simulink model "three_b_attitude_control_rotationMatrix"  (R2021a)
settings: Solver=ode23t  StartTime=0.0  StopTime=100  RelTol=1e-5
undefined symbols (not defined in the file): eul_init, g, I, km, kt, L, m, pm_0, sigbuilder_block, thrust_max, TQ_max_per_motor, Vb_init, Vm_0, wb_init, Xe_init, xme_0
libraries: simulink_extras x18, sharedtransform x3, simulink x1
(part 1 of 2)
settings Model: Creator=Petronas-Tareq  LastModifiedBy=Petronas-Tareq

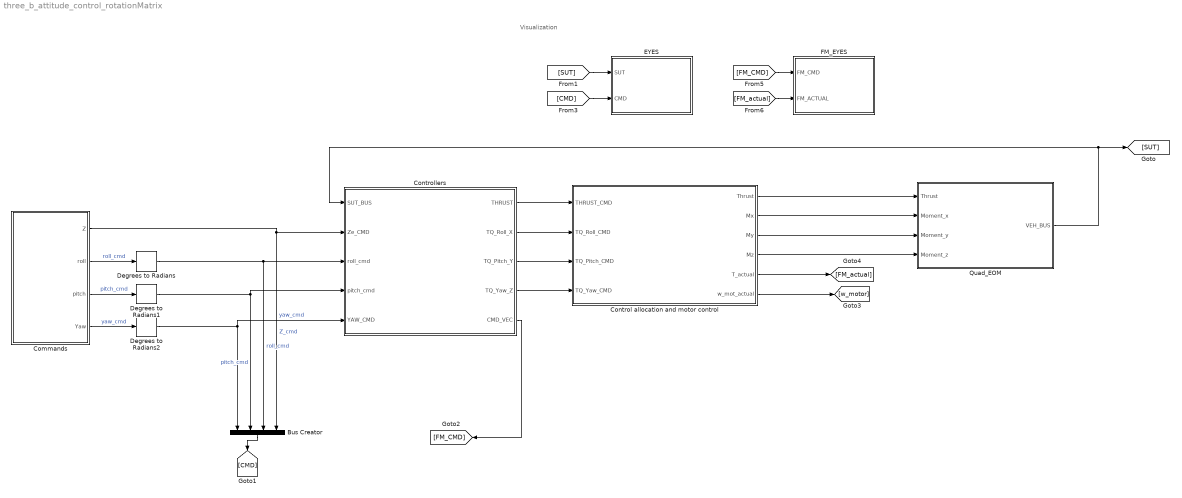
== system three_b_attitude_control_rotationMatrix ==
  note: Visualization
  Bus Creator : BusCreator  Inputs=4
  Commands : Subsystem  Variant=on  VariantControlMode=label  LabelModeActiveChoice=Choice_5
  Control allocation and motor control : Subsystem  Variant=on  VariantControlMode=label  LabelModeActiveChoice=Choice2
      mask Display: image('$imagefile'); % Use "Edit Image" on toolstrip to change.
  Controllers : Subsystem
      mask Display: image('$imagefile'); % Use "Edit Image" on toolstrip to change.
  Degrees to Radians : simulink_extras/Transformations/Degrees to Radians
  Degrees to Radians1 : simulink_extras/Transformations/Degrees to Radians
  Degrees to Radians2 : simulink_extras/Transformations/Degrees to Radians
  EYES : Subsystem
  FM_EYES : Subsystem
  Quad_EOM : Subsystem
      mask Display: image('$imagefile'); % Use "Edit Image" on toolstrip to change.
  wires:
  [FM_CMD] -> FM_EYES/1(FM_CMD)
  Controllers/5(CMD_VEC) -> [FM_CMD]
  [FM_actual] -> FM_EYES/2(FM_ACTUAL)
  Commands/1(Z) -> Bus Creator/4, Controllers/2(Ze_CMD)  "Z_cmd"
  Degrees to Radians/1 -> Bus Creator/3, Controllers/3(roll_cmd)  "roll_cmd"
  Degrees to Radians2/1 -> Bus Creator/1, Controllers/5(YAW_CMD)  "yaw_cmd"
  [SUT] -> EYES/1(SUT)
  [CMD] -> EYES/2(CMD)
  Bus Creator/1 -> [CMD]
  Degrees to Radians1/1 -> Bus Creator/2, Controllers/4(pitch_cmd)  "pitch_cmd"
  Commands/2(roll) -> Degrees to Radians/1  "roll_cmd"
  Commands/3(pitch) -> Degrees to Radians1/1  "pitch_cmd"
  Commands/4(Yaw) -> Degrees to Radians2/1  "yaw_cmd"
  Controllers/1(THRUST) -> Control allocation and motor control/1(THRUST_CMD)
  Controllers/2(TQ_Roll_X) -> Control allocation and motor control/2(TQ_Roll_CMD)
  Controllers/3(TQ_Pitch_Y) -> Control allocation and motor control/3(TQ_Pitch_CMD)
  Controllers/4(TQ_Yaw_Z) -> Control allocation and motor control/4(TQ_Yaw_CMD)
  Control allocation and motor control/1(Thrust) -> Quad_EOM/1(Thrust)
  Control allocation and motor control/2(Mx) -> Quad_EOM/2(Moment_x)
  Control allocation and motor control/3(My) -> Quad_EOM/3(Moment_y)
  Control allocation and motor control/4(Mz) -> Quad_EOM/4(Moment_z)
  Control allocation and motor control/5(T_actual) -> [FM_actual]
  Control allocation and motor control/6(w_mot_actual) -> [w_motor]
  Quad_EOM/1(VEH_BUS) -> [SUT], Controllers/1(SUT_BUS)

== system three_b_attitude_control_rotationMatrix/Commands ==
  note: 1) Add Subsystem or Model blocks as valid variant choices.
      | 2) You cannot connect blocks at this level. At simulation, connectivity is automatically
      | determined, based on the active variant and port name matching.
  "Altitude " : Subsystem  Tag=STV Subsys  LoadFcn=sigbuilder_block('load');  StartFcn=sigbuilder_block('start');  StopFcn=sigbuilder_block('stop');  ClipboardFcn=sigbuilder_block('clipboard');  VariantControl=Choice_1  mask(Sigbuilder block){tuvar=[0:10]}
      mask help: Simulink:masks:SigbuilderBlock_MD
      mask init:
      | if ~strcmp(get_param(bdroot(gcbh),'SimulationStatus'),'stopped') tuvar = sigbuilder_block('maskInit'); end
      settings: CopyFcn=sigbuilder_block('copy');  DeleteFcn=sigbuilder_block('delete');  ModelCloseFcn=sigbuilder_block('modelClose');  PreSaveFcn=sigbuilder_block('preSave');  PauseFcn=sigbuilder_block('pause');  ContinueFcn=sigbuilder_block('continue');  NameChangeFcn=sigbuilder_block('namechange');  OpenFcn=sigbuilder_block('open',[200.1 155.1 551.4 400.5 ]);  CloseFcn=sigbuilder_block('close');
      mask Display: plot(0, 0, 100, 100,[2, 2, 32, 32, 2], [68, 8, 8, 68, 68],[32, 2], [38, 38], [32, 19, 2],[53, 60, 44], [32, 17, 17, 2],[16, 16, 31, 31]);txt = getActiveGroup(gcbh);text(2, 100, txt,'verticalAlignment', 'top');
  Ground : Subsystem  Tag=STV Subsys  LoadFcn=sigbuilder_block('load');  StartFcn=sigbuilder_block('start');  StopFcn=sigbuilder_block('stop');  ClipboardFcn=sigbuilder_block('clipboard');  VariantControl=Choice  mask(Sigbuilder block){tuvar=[0:10]}
      mask help: Simulink:masks:SigbuilderBlock_MD
      mask init:
      | if ~strcmp(get_param(bdroot(gcbh),'SimulationStatus'),'stopped') tuvar = sigbuilder_block('maskInit'); end
      settings: CopyFcn=sigbuilder_block('copy');  DeleteFcn=sigbuilder_block('delete');  ModelCloseFcn=sigbuilder_block('modelClose');  PreSaveFcn=sigbuilder_block('preSave');  PauseFcn=sigbuilder_block('pause');  ContinueFcn=sigbuilder_block('continue');  NameChangeFcn=sigbuilder_block('namechange');  OpenFcn=sigbuilder_block('open',[200.1 155.1 551.4 400.5 ]);  CloseFcn=sigbuilder_block('close');
      mask Display: plot(0, 0, 100, 100,[2, 2, 32, 32, 2], [68, 8, 8, 68, 68],[32, 2], [38, 38], [32, 19, 2],[53, 60, 44], [32, 17, 17, 2],[16, 16, 31, 31]);txt = getActiveGroup(gcbh);text(2, 100, txt,'verticalAlignment', 'top');
  Pitch : Subsystem  Tag=STV Subsys  LoadFcn=sigbuilder_block('load');  StartFcn=sigbuilder_block('start');  StopFcn=sigbuilder_block('stop');  ClipboardFcn=sigbuilder_block('clipboard');  VariantControl=Choice_3  mask(Sigbuilder block){tuvar=[0:10]}
      mask help: Simulink:masks:SigbuilderBlock_MD
      mask init:
      | if ~strcmp(get_param(bdroot(gcbh),'SimulationStatus'),'stopped') tuvar = sigbuilder_block('maskInit'); end
      settings: CopyFcn=sigbuilder_block('copy');  DeleteFcn=sigbuilder_block('delete');  ModelCloseFcn=sigbuilder_block('modelClose');  PreSaveFcn=sigbuilder_block('preSave');  PauseFcn=sigbuilder_block('pause');  ContinueFcn=sigbuilder_block('continue');  NameChangeFcn=sigbuilder_block('namechange');  OpenFcn=sigbuilder_block('open',[452.4 149.7 551.4 400.5 ]);  CloseFcn=sigbuilder_block('close');
      mask Display: plot(0, 0, 100, 100,[2, 2, 32, 32, 2], [68, 8, 8, 68, 68],[32, 2], [38, 38], [32, 19, 2],[53, 60, 44], [32, 17, 17, 2],[16, 16, 31, 31]);txt = getActiveGroup(gcbh);text(2, 100, txt,'verticalAlignment', 'top');
  Roll : Subsystem  Tag=STV Subsys  LoadFcn=sigbuilder_block('load');  StartFcn=sigbuilder_block('start');  StopFcn=sigbuilder_block('stop');  ClipboardFcn=sigbuilder_block('clipboard');  VariantControl=Choice_2  mask(Sigbuilder block){tuvar=[0:10]}
      mask help: Simulink:masks:SigbuilderBlock_MD
      mask init:
      | if ~strcmp(get_param(bdroot(gcbh),'SimulationStatus'),'stopped') tuvar = sigbuilder_block('maskInit'); end
      settings: CopyFcn=sigbuilder_block('copy');  DeleteFcn=sigbuilder_block('delete');  ModelCloseFcn=sigbuilder_block('modelClose');  PreSaveFcn=sigbuilder_block('preSave');  PauseFcn=sigbuilder_block('pause');  ContinueFcn=sigbuilder_block('continue');  NameChangeFcn=sigbuilder_block('namechange');  OpenFcn=sigbuilder_block('open',[452.4 149.7 551.4 400.5 ]);  CloseFcn=sigbuilder_block('close');
      mask Display: plot(0, 0, 100, 100,[2, 2, 32, 32, 2], [68, 8, 8, 68, 68],[32, 2], [38, 38], [32, 19, 2],[53, 60, 44], [32, 17, 17, 2],[16, 16, 31, 31]);txt = getActiveGroup(gcbh);text(2, 100, txt,'verticalAlignment', 'top');
  multisteps : Subsystem  Tag=STV Subsys  LoadFcn=sigbuilder_block('load');  StartFcn=sigbuilder_block('start');  StopFcn=sigbuilder_block('stop');  ClipboardFcn=sigbuilder_block('clipboard');  VariantControl=Choice_5  mask(Sigbuilder block){tuvar=[0:10]}
      mask help: Simulink:masks:SigbuilderBlock_MD
      mask init:
      | if ~strcmp(get_param(bdroot(gcbh),'SimulationStatus'),'stopped') tuvar = sigbuilder_block('maskInit'); end
      settings: CopyFcn=sigbuilder_block('copy');  DeleteFcn=sigbuilder_block('delete');  ModelCloseFcn=sigbuilder_block('modelClose');  PreSaveFcn=sigbuilder_block('preSave');  PauseFcn=sigbuilder_block('pause');  ContinueFcn=sigbuilder_block('continue');  NameChangeFcn=sigbuilder_block('namechange');  OpenFcn=sigbuilder_block('open',[200.1 155.1 551.4 400.5 ]);  CloseFcn=sigbuilder_block('close');
      mask Display: plot(0, 0, 100, 100,[2, 2, 32, 32, 2], [68, 8, 8, 68, 68],[32, 2], [38, 38], [32, 19, 2],[53, 60, 44], [32, 17, 17, 2],[16, 16, 31, 31]);txt = getActiveGroup(gcbh);text(2, 100, txt,'verticalAlignment', 'top');
  yaw : Subsystem  Tag=STV Subsys  LoadFcn=sigbuilder_block('load');  StartFcn=sigbuilder_block('start');  StopFcn=sigbuilder_block('stop');  ClipboardFcn=sigbuilder_block('clipboard');  VariantControl=Choice_4  mask(Sigbuilder block){tuvar=[0:10]}
      mask help: Simulink:masks:SigbuilderBlock_MD
      mask init:
      | if ~strcmp(get_param(bdroot(gcbh),'SimulationStatus'),'stopped') tuvar = sigbuilder_block('maskInit'); end
      settings: CopyFcn=sigbuilder_block('copy');  DeleteFcn=sigbuilder_block('delete');  ModelCloseFcn=sigbuilder_block('modelClose');  PreSaveFcn=sigbuilder_block('preSave');  PauseFcn=sigbuilder_block('pause');  ContinueFcn=sigbuilder_block('continue');  NameChangeFcn=sigbuilder_block('namechange');  OpenFcn=sigbuilder_block('open',[452.4 149.7 551.4 400.5 ]);  CloseFcn=sigbuilder_block('close');
      mask Display: plot(0, 0, 100, 100,[2, 2, 32, 32, 2], [68, 8, 8, 68, 68],[32, 2], [38, 38], [32, 19, 2],[53, 60, 44], [32, 17, 17, 2],[16, 16, 31, 31]);txt = getActiveGroup(gcbh);text(2, 100, txt,'verticalAlignment', 'top');
  Z : Outport
  roll : Outport  Port=2
  pitch : Outport  Port=3
  Yaw : Outport  Port=4

== system three_b_attitude_control_rotationMatrix/Control allocation and motor control ==
  note: 1) Add Subsystem or Model blocks as valid variant choices.
      | 2) You cannot connect blocks at this level. At simulation, connectivity is automatically
      | determined, based on the active variant and port name matching.
  THRUST_CMD : Inport
  TQ_Roll_CMD : Inport  Port=2
  TQ_Pitch_CMD : Inport  Port=3
  TQ_Yaw_CMD : Inport  Port=4
  Ideal Actuators with allocation : Subsystem  VariantControl=Choice2
  Ideal Actuattion (direct transfer) : Subsystem  VariantControl=Choice1
  Thrust : Outport
  Mx : Outport  Port=2
  My : Outport  Port=3
  Mz : Outport  Port=4
  T_actual : Outport  Port=5
  w_mot_actual : Outport  Port=6

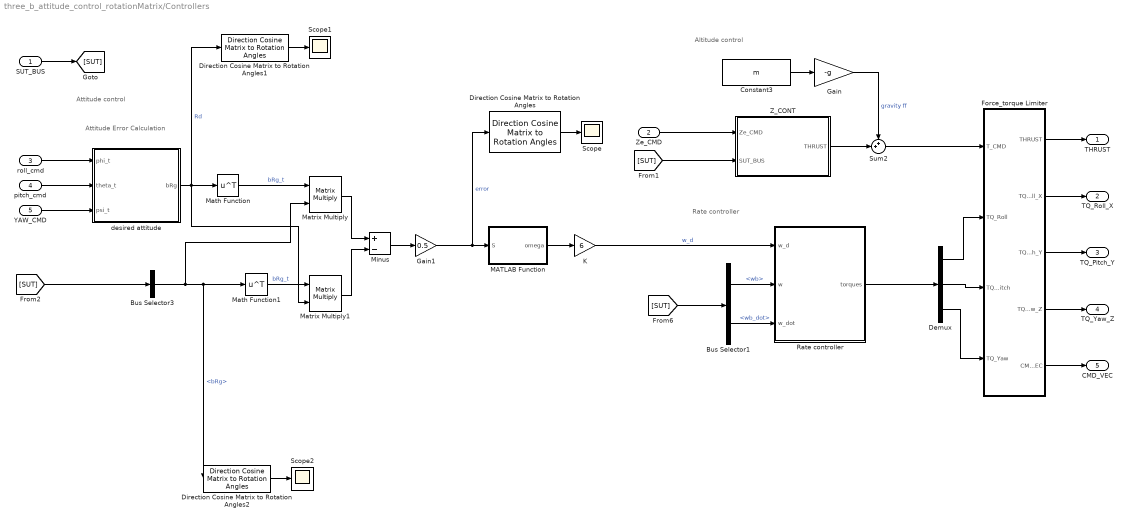
== system three_b_attitude_control_rotationMatrix/Controllers ==
  note: Rate controller
  note: Altitude control
  note: Attitude control
  note: Attitude Error Calculation
  SUT_BUS : Inport
  Ze_CMD : Inport  Port=2
  roll_cmd : Inport  Port=3
  pitch_cmd : Inport  Port=4
  YAW_CMD : Inport  Port=5
  Bus Selector1 : BusSelector  OutputSignals=wb,wb_dot
  Bus Selector3 : BusSelector  OutputSignals=bRg
  Constant3 : Constant  Value=m
  Demux : Demux  Outputs=3
  Direction Cosine Matrix to Rotation Angles : sharedtransform/Direction Cosine Matrix to Rotation Angles  rotationOrder=ZYX  aMode=aMode  action=None  tolerance=eps(2)
      settings: SourceProductBaseCode=AE,PW,DR,MT,UV,VE
  Direction Cosine Matrix to Rotation Angles1 : sharedtransform/Direction Cosine Matrix to Rotation Angles  rotationOrder=ZYX  aMode=aMode  action=None  tolerance=eps(2)
      settings: SourceProductBaseCode=AE,PW,DR,MT,UV,VE
  Direction Cosine Matrix to Rotation Angles2 : sharedtransform/Direction Cosine Matrix to Rotation Angles  rotationOrder=ZYX  aMode=aMode  action=None  tolerance=eps(2)
      settings: SourceProductBaseCode=AE,PW,DR,MT,UV,VE
  Force_torque Limiter : Subsystem
  Gain : Gain  Gain=-g
  Gain1 : Gain  Gain=0.5
  K : Gain  Gain=6
  MATLAB Function : MATLAB Function  TreatAsAtomicUnit=on
  Math Function : Math  Operator=transpose  SignedPower=on  SaturateOnIntegerOverflow=on
  Math Function1 : Math  Operator=transpose  SignedPower=on  SaturateOnIntegerOverflow=on
  Matrix Multiply : Product  Multiplication=Matrix(*)
  Matrix Multiply1 : Product  Multiplication=Matrix(*)
  Minus : Sum  Inputs=+-
  Rate controller : Subsystem
  Scope : Scope
  Scope1 : Scope
  Scope2 : Scope
  Sum2 : Sum  Inputs=++|
  Z_CONT : Subsystem
  desired attitude : MATLAB Function  TreatAsAtomicUnit=on
  THRUST : Outport  VectorParamsAs1DForOutWhenUnconnected=off
  TQ_Roll_X : Outport  Port=2  VectorParamsAs1DForOutWhenUnconnected=off
  TQ_Pitch_Y : Outport  Port=3  VectorParamsAs1DForOutWhenUnconnected=off
  TQ_Yaw_Z : Outport  Port=4  VectorParamsAs1DForOutWhenUnconnected=off
  CMD_VEC : Outport  Port=5  VectorParamsAs1DForOutWhenUnconnected=off
  wires:
  SUT_BUS/1 -> [SUT]
  Ze_CMD/1 -> Z_CONT/1(Ze_CMD)
  YAW_CMD/1 -> desired attitude/3(psi_t)
  Z_CONT/1(THRUST) -> Sum2/2
  Sum2/1 -> Force_torque Limiter/1(T_CMD)
  Force_torque Limiter/1(THRUST) -> THRUST/1
  Force_torque Limiter/2(TQ_Roll_X) -> TQ_Roll_X/1
  Force_torque Limiter/3(TQ_Pitch_Y) -> TQ_Pitch_Y/1
  Force_torque Limiter/4(TQ_Yaw_Z) -> TQ_Yaw_Z/1
  Force_torque Limiter/5(CMD_VEC) -> CMD_VEC/1
  Gain/1 -> Sum2/1  "gravity ff"
  Constant3/1 -> Gain/1
  pitch_cmd/1 -> desired attitude/2(theta_t)
  roll_cmd/1 -> desired attitude/1(phi_t)
  desired attitude/1(bRg) -> Direction Cosine Matrix to Rotation Angles1/1, Math Function/1, Matrix Multiply1/2  "Rd"
  [SUT] -> Z_CONT/2(SUT_BUS)
  [SUT] -> Bus Selector3/1
  Bus Selector3/1 -> Matrix Multiply/2, Direction Cosine Matrix to Rotation Angles2/1, Math Function1/1  "<bRg>"
  Math Function/1 -> Matrix Multiply/1  "bRg_t"
  Math Function1/1 -> Matrix Multiply1/1  "bRg_t"
  Minus/1 -> Gain1/1
  Matrix Multiply/1 -> Minus/1
  Matrix Multiply1/1 -> Minus/2
  Gain1/1 -> Direction Cosine Matrix to Rotation Angles/1, MATLAB Function/1(S)  "error"
  MATLAB Function/1(omega) -> K/1
  [SUT] -> Bus Selector1/1
  K/1 -> Rate controller/1(w_d)  "w_d"
  Bus Selector1/1 -> Rate controller/2(w)  "<wb>"
  Bus Selector1/2 -> Rate controller/3(w_dot)  "<wb_dot>"
  Rate controller/1(torques) -> Demux/1
  Demux/1 -> Force_torque Limiter/2(TQ_Roll)
  Demux/2 -> Force_torque Limiter/3(TQ_Pitch)
  Demux/3 -> Force_torque Limiter/4(TQ_Yaw)
  Direction Cosine Matrix to Rotation Angles/1 -> Scope/1
  Direction Cosine Matrix to Rotation Angles1/1 -> Scope1/1
  Direction Cosine Matrix to Rotation Angles2/1 -> Scope2/1

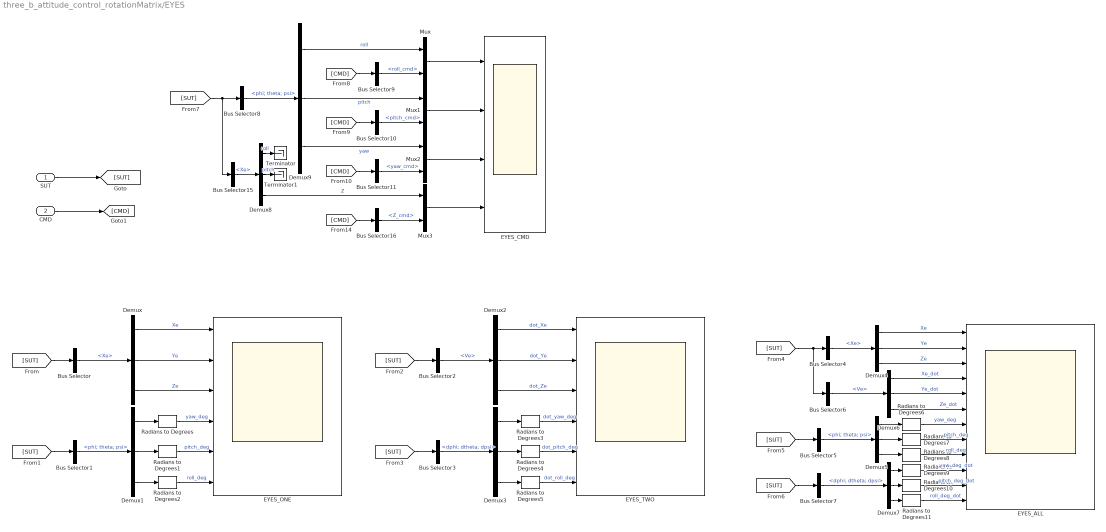
== system three_b_attitude_control_rotationMatrix/EYES ==
  SUT : Inport
  CMD : Inport  Port=2
  Bus Selector : BusSelector  OutputSignals=Xe
  Bus Selector1 : BusSelector  OutputSignals=phi; theta; psi
  Bus Selector10 : BusSelector  OutputSignals=pitch_cmd
  Bus Selector11 : BusSelector  OutputSignals=yaw_cmd
  Bus Selector15 : BusSelector  OutputSignals=Xe
  Bus Selector16 : BusSelector  OutputSignals=Z_cmd
  Bus Selector2 : BusSelector  OutputSignals=Ve
  Bus Selector3 : BusSelector  OutputSignals=dphi; dtheta; dpsi
  Bus Selector4 : BusSelector  OutputSignals=Xe
  Bus Selector5 : BusSelector  OutputSignals=phi; theta; psi
  Bus Selector6 : BusSelector  OutputSignals=Ve
  Bus Selector7 : BusSelector  OutputSignals=dphi; dtheta; dpsi
  Bus Selector8 : BusSelector  OutputSignals=phi; theta; psi
  Bus Selector9 : BusSelector  OutputSignals=roll_cmd
  Demux{,1..9} (10 alike) : Demux  Outputs=3
  EYES_ALL : Scope  NumInputPorts=12
  EYES_CMD : Scope  NumInputPorts=4
  EYES_ONE : Scope  NumInputPorts=6
  EYES_TWO : Scope  NumInputPorts=6
  Mux{,1..3} (4 alike) : Mux  Inputs=2
  Radians to Degrees{,1..11} (12 alike) : simulink_extras/Transformations/Radians to Degrees
  Terminator : Terminator
  Terminator1 : Terminator
  wires:
  SUT/1 -> [SUT]
  [SUT] -> Bus Selector/1
  Demux/2 -> EYES_ONE/2  "Ye"
  Demux/3 -> EYES_ONE/3  "Ze"
  Demux/1 -> EYES_ONE/1  "Xe"
  Bus Selector/1 -> Demux/1  "<Xe>"
  Bus Selector1/1 -> Demux1/1  "<phi; theta; psi>"
  [SUT] -> Bus Selector1/1
  Demux1/1 -> Radians to Degrees/1
  Radians to Degrees/1 -> EYES_ONE/4  "yaw_deg"
  Radians to Degrees1/1 -> EYES_ONE/5  "pitch_deg"
  Radians to Degrees2/1 -> EYES_ONE/6  "roll_deg"
  Demux1/3 -> Radians to Degrees2/1
  Demux1/2 -> Radians to Degrees1/1
  [SUT] -> Bus Selector2/1
  Demux2/2 -> EYES_TWO/2  "dot_Ye"
  Demux2/3 -> EYES_TWO/3  "dot_Ze"
  Demux2/1 -> EYES_TWO/1  "dot_Xe"
  Bus Selector2/1 -> Demux2/1  "<Ve>"
  Bus Selector3/1 -> Demux3/1  "<dphi; dtheta; dpsi>"
  [SUT] -> Bus Selector3/1
  Demux3/1 -> Radians to Degrees3/1
  Radians to Degrees3/1 -> EYES_TWO/4  "dot_yaw_deg"
  Radians to Degrees4/1 -> EYES_TWO/5  "dot_pitch_deg"
  Radians to Degrees5/1 -> EYES_TWO/6  "dot_roll_deg"
  Demux3/3 -> Radians to Degrees5/1
  Demux3/2 -> Radians to Degrees4/1
  [SUT] -> Bus Selector6/1, Bus Selector4/1
  Demux4/2 -> EYES_ALL/2  "Ye"
  Demux4/3 -> EYES_ALL/3  "Ze"
  Demux4/1 -> EYES_ALL/1  "Xe"
  Bus Selector4/1 -> Demux4/1  "<Xe>"
  Bus Selector5/1 -> Demux5/1  "<phi; theta; psi>"
  [SUT] -> Bus Selector5/1
  Demux5/1 -> Radians to Degrees6/1
  Demux6/1 -> EYES_ALL/4  "Xe_dot"
  Demux6/2 -> EYES_ALL/5  "Ye_dot"
  Demux6/3 -> EYES_ALL/6  "Ze_dot"
  Demux5/3 -> Radians to Degrees8/1
  Demux5/2 -> Radians to Degrees7/1
  Bus Selector6/1 -> Demux6/1  "<Ve>"
  Radians to Degrees6/1 -> EYES_ALL/7  "yaw_deg"
  Radians to Degrees7/1 -> EYES_ALL/8  "pitch_deg"
  Radians to Degrees8/1 -> EYES_ALL/9  "roll_deg"
  Bus Selector7/1 -> Demux7/1  "<dphi; dtheta; dpsi>"
  [SUT] -> Bus Selector7/1
  Demux7/1 -> Radians to Degrees9/1
  Demux7/2 -> Radians to Degrees10/1
  Demux7/3 -> Radians to Degrees11/1
  Radians to Degrees9/1 -> EYES_ALL/10  "yaw_deg_dot"
  Radians to Degrees10/1 -> EYES_ALL/11  "pitch_deg_dot"
  Radians to Degrees11/1 -> EYES_ALL/12  "roll_deg_dot"
  CMD/1 -> [CMD]
  [SUT] -> Bus Selector8/1, Bus Selector15/1
  Demux9/2 -> Mux1/1  "pitch"
  Demux9/1 -> Mux/1  "roll"
  Bus Selector8/1 -> Demux9/1  "<phi; theta; psi>"
  Mux/1 -> EYES_CMD/1
  Mux1/1 -> EYES_CMD/2
  Mux2/1 -> EYES_CMD/3
  Demux9/3 -> Mux2/1  "yaw"
  [CMD] -> Bus Selector9/1
  Bus Selector9/1 -> Mux/2  "<roll_cmd>"
  [CMD] -> Bus Selector10/1
  Bus Selector10/1 -> Mux1/2  "<pitch_cmd>"
  [CMD] -> Bus Selector11/1
  Bus Selector11/1 -> Mux2/2  "<yaw_cmd>"
  Bus Selector15/1 -> Demux8/1  "<Xe>"
  Demux8/1 -> Terminator/1  "roll"
  Demux8/2 -> Terminator1/1  "pitch"
  Bus Selector16/1 -> Mux3/2  "<Z_cmd>"
  [CMD] -> Bus Selector16/1
  Mux3/1 -> EYES_CMD/4
  Demux8/3 -> Mux3/1  "Z"

== system three_b_attitude_control_rotationMatrix/FM_EYES ==
  FM_CMD : Inport
  FM_ACTUAL : Inport  Port=2
  FM CMD vs Actual : Scope  NumInputPorts=4
  FM_Mux : Subsystem
  wires:
  FM_CMD/1 -> [FM_CMD]
  [FM_CMD] -> FM_Mux/1(FM_CMD)
  [FM] -> FM_Mux/2(FM)
  FM_Mux/1(Y1) -> FM CMD vs Actual/1  "Thrust"
  FM_Mux/2(Y2) -> FM CMD vs Actual/2  "TQ_Roll_X"
  FM_Mux/3(w3) -> FM CMD vs Actual/3  "TQ_Pitch_Y"
  FM_Mux/4(Y4) -> FM CMD vs Actual/4  "TQ_Yaw_Z"
  FM_ACTUAL/1 -> [FM]

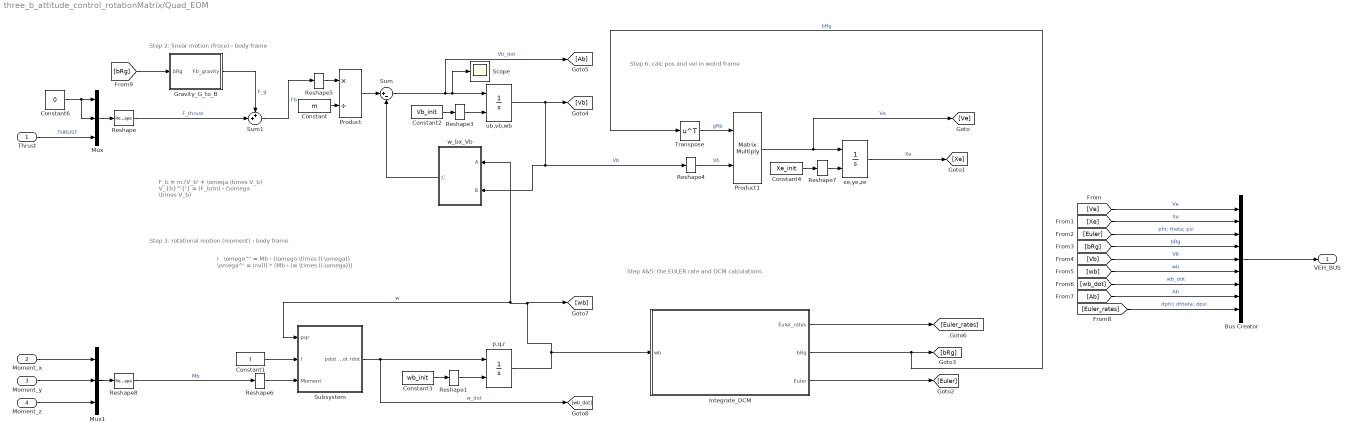
== system three_b_attitude_control_rotationMatrix/Quad_EOM ==
  note: Step 3: rotational motion (moment) - body frame
  note: F_b = m.(V_b' + \omega \times V_b)
      |
      | V_{b}^{'} = (F_b/m) - (\omega \times V_b)
  note: Step 2: linear motion (froce) - body frame
  note: Step 6: calc pos and vel in wolrd frame
  note: I . \omega^' = Mb - (\omega \times (I.\omega))
      |
      | \omega^' = inv(I) * (Mb - (w \times (I.\omega)))
  note: Step 4&5: the EULER rate and DCM calculations
  Thrust : Inport
  Moment_x : Inport  Port=2
  Moment_y : Inport  Port=3
  Moment_z : Inport  Port=4
  Bus Creator : BusCreator  Inputs=9
  Constant : Constant  Value=m  OutDataTypeStr=Inherit: Inherit via back propagation
  Constant1 : Constant  Value=I  OutDataTypeStr=Inherit: Inherit via back propagation
  Constant2 : Constant  Value=Vb_init  OutDataTypeStr=Inherit: Inherit via back propagation
  Constant3 : Constant  Value=wb_init  OutDataTypeStr=Inherit: Inherit via back propagation
  Constant4 : Constant  Value=Xe_init  OutDataTypeStr=Inherit: Inherit via back propagation
  Constant6 : Constant  Value=0
  Gravity_G_to_B : Subsystem
  Integrate_DCM : Subsystem
  Mux : Mux  Inputs=3
  Mux1 : Mux  Inputs=3
  Product : Product  Inputs=*/  SaturateOnIntegerOverflow=on  OutDataTypeStr=Inherit: Same as first input
  Product1 : Product  Multiplication=Matrix(*)  InputSameDT=on  SaturateOnIntegerOverflow=on  OutDataTypeStr=Inherit: Same as first input
  Reshape{,1,3..8} (8 alike) : Reshape  OutputDimensionality=Column vector (2-D)
  Scope : Scope
  Subsystem : Subsystem
  Sum : Sum  Inputs=|+-  SaturateOnIntegerOverflow=on
  Sum1 : Sum  Inputs=++|
  Transpose : Math  Operator=transpose  SignedPower=on  SaturateOnIntegerOverflow=on
  "p,q,r " : Integrator  InitialConditionSource=external  InitialCondition=pm_0
  ub,vb,wb : Integrator  InitialConditionSource=external  InitialCondition=Vm_0
  w_bx_Vb : Subsystem
      mask Display:
      | text(.5,.5,'Cross\nProduct\n\nC = AxB', ...
      | 	'HorizontalAlignment','Center',...
      | 	'VerticalAlignment','middle')
  xe,ye,ze : Integrator  InitialConditionSource=external  InitialCondition=xme_0
  VEH_BUS : Outport  VectorParamsAs1DForOutWhenUnconnected=off
  wires:
  [Euler] -> Bus Creator/3  "phi; theta; psi"
  [Xe] -> Bus Creator/2  "Xe"
  [Ve] -> Bus Creator/1  "Ve"
  [bRg] -> Bus Creator/4  "bRg"
  [Ab] -> Bus Creator/8  "Ab"
  [wb_dot] -> Bus Creator/7  "wb_dot"
  Bus Creator/1 -> VEH_BUS/1
  [Vb] -> Bus Creator/5  "Vb"
  [wb] -> Bus Creator/6  "wb"
  [Euler_rates] -> Bus Creator/9  "dphi; dtheta; dpsi"
  Reshape8/1 -> Reshape6/1  "Mb"
  Reshape6/1 -> Subsystem/3(Moment)
  Reshape1/1 -> "p,q,r "/2
  Transpose/1 -> Product1/1  "gRb"
  Constant2/1 -> Reshape3/1
  Subsystem/1(pdot qdot rdot) -> [wb_dot], "p,q,r "/1  "w_dot"
  Constant/1 -> Product/2
  Constant1/1 -> Subsystem/2(I)
  Reshape4/1 -> Product1/2  "Vb"
  w_bx_Vb/1(C) -> Sum/2
  Integrate_DCM/2(bRg) -> [bRg], Transpose/1  "bRg"
  Sum/1 -> [Ab], Scope/1, ub,vb,wb/1  "Vb_dot"
  Constant4/1 -> Reshape7/1
  Reshape3/1 -> ub,vb,wb/2
  Reshape7/1 -> xe,ye,ze/2
  Product1/1 -> [Ve], xe,ye,ze/1  "Ve"
  Reshape5/1 -> Product/1
  xe,ye,ze/1 -> [Xe]  "Xe"
  Sum1/1 -> Reshape5/1  "Fb"
  Constant3/1 -> Reshape1/1
  Product/1 -> Sum/1
  Constant6/1 -> Mux/2, Mux/1
  Gravity_G_to_B/1(Fb_gravity) -> Sum1/1  "F_g"
  Mux/1 -> Reshape/1
  Reshape/1 -> Sum1/2  "F_thrust"
  Thrust/1 -> Mux/3  "THRUST"
  [bRg] -> Gravity_G_to_B/1(bRg)
  Moment_y/1 -> Mux1/2
  Moment_z/1 -> Mux1/3
  Mux1/1 -> Reshape8/1
  Moment_x/1 -> Mux1/1
  "p,q,r "/1 -> [wb], Subsystem/1(pqr), w_bx_Vb/1(A), Integrate_DCM/1(wb)  "w"
  ub,vb,wb/1 -> [Vb], w_bx_Vb/2(B), Reshape4/1  "Vb"
  Integrate_DCM/1(Euler_rates) -> [Euler_rates]
  Integrate_DCM/3(Euler) -> [Euler]

== system three_b_attitude_control_rotationMatrix/Commands/Altitude  ==
  Demux : Demux  Tag=STV Demux
      settings: DisplayOption=none
  FromWs : FromWorkspace  Tag=STV FromWs  VariableName=tuvar
      SigBuilderData=|
      | common.afterFinalStr = 'Extrapolate'
      | common.sampleTime = 0
      | dataSet(1).timeRange = [0 200]
      | dataSet(1).name = 'small_steps'
      | dataSet(2).timeRange = [0 200]
      | dataSet(2).name = 'zStairs_xyConstVEL'
      | dataSet(3).timeRange = [0 500]
      | dataSet(3).name = 'sineWaves'
      | dataSet(4).timeRange = [0 200]
      | dataSet(4).name = 'ZERO'
      | dataSet(5).timeRange = [0 200]
      | dataSet(5).name = 'SEARCH_P1'
      | sbobj.Name = 'Signal Builder'
      | sbobj.Groups(1).Name = 'small_steps'
      | sbobj.Groups(1).Signals(1).Name = 'Z'
      | sbobj.Groups(1).Signals(1).XData = [0 10 10.000001 20 20.000001 30 30.000001 55 200]
      | sbobj.Groups(1).Signals(1).YData = [0 0 2 2 2 2 2 2 2]
      | sbobj.Groups(1).Signals(2).Name = 'roll'
      | sbobj.Groups(1).Signals(2).XData = [0 10 10.000001 20 20.000001 30 30.000001 55 200]
      | sbobj.Groups(1).Signals(2).YData = [0 0 0 0 3 3 3 3 3]
      | sbobj.Groups(1).Signals(3).Name = 'pitch'
      | sbobj.Groups(1).Signals(3).XData = [0 10 10.000001 20 20.000001 30 30.000001 55 200]
      | sbobj.Groups(1).Signals(3).YData = [0 0 0 0 0 0 1 1 1]
      | sbobj.Groups(1).Signals(4).Name = 'Yaw'
      | sbobj.Groups(1).Signals(4).XData = [0 200]
      | sbobj.Groups(1).Signals(4).YData = [0 0]
      | sbobj.Groups(1).TimeRange = [0 200]
      | sbobj.Groups(2).Name = 'zStairs_xyConstVEL'
      | sbobj.Groups(2).Signals(1).Name = 'Z'
      | sbobj.Groups(2).Signals(1).XData = [0 10 10.000001 20 20.000001 30 30.000001 40 40.000001 55 200]
      | sbobj.Groups(2).Signals(1).YData = [0 0 1 1 2 2 1 1 0 0 0]
      | sbobj.Groups(2).Signals(2).Name = 'roll'
      | sbobj.Groups(2).Signals(2).XData = [0 10 10.000001 20 20.000001 30 30.000001 40 40.000001 55 200]
      | sbobj.Groups(2).Signals(2).YData = [0 1 1.0000001 2 2.0000001 3 3.0000001 4 4.0000001 5.5 20]
      | sbobj.Groups(2).Signals(3).Name = 'pitch'
      | sbobj.Groups(2).Signals(3).XData = [0 10 10.000001 20 20.000001 30 30.000001 40 40.000001 55 200]
      | sbobj.Groups(2).Signals(3).YData = [0 0.5 0.50000005 1 1.00000005 1.5 1.50000005 2 2.00000005 2.75 10]
      | sbobj.Groups(2).Signals(4).Name = 'Yaw'
      | sbobj.Groups(2).Signals(4).XData = [0 200]
      | sbobj.Groups(2).Signals(4).YData = [0 0]
      | sbobj.Groups(2).TimeRange = [0 200]
      | sbobj.Groups(3).Name = 'sineWaves'
      | sbobj.Groups(3).Signals(1).Name = 'Z'
      | sbobj.Groups(3).Signals(1).XData = [0 0.1 0.2 0.3 0.4 0.5 0.6 0.7 0.8 0.9 1 1.1 ... (5001 elements, 1x5001)]
      | sbobj.Groups(3).Signals(1).YData = [0 0.0314107325553 0.0627904665622 0.0941082340641 0.125333128258 0.156434333994 0.18738115819 0.218143060119 0.248689681547 0.278990876699 0.309016742004 0.338737645607 ... (5001 elements, 1x5001)]
      | sbobj.Groups(3).Signals(2).Name = 'roll'
      | sbobj.Groups(3).Signals(2).XData = [0 0.1 0.2 0.3 0.4 0.5 0.6 0.7 0.8 0.9 1 1.1 ... (5001 elements, 1x5001)]
      | sbobj.Groups(3).Signals(2).YData = [0 0.01 0.02 0.03 0.04 0.05 0.06 0.07 0.08 0.09 0.1 0.11 ... (5001 elements, 1x5001)]
      | sbobj.Groups(3).Signals(3).Name = 'pitch'
      | sbobj.Groups(3).Signals(3).XData = [0 0.1 0.2 0.3 0.4 0.5 0.6 0.7 0.8 0.9 1 1.1 ... (5001 elements, 1x5001)]
      | sbobj.Groups(3).Signals(3).YData = [0 0.0157073040455 0.0314107325553 0.04710641095 0.0627904665622 0.0784590295926 0.0941082340641 0.109734218776 0.125333128258 0.140901113717 0.156434333994 0.171928956505 ... (5001 elements, 1x5001)]
      | sbobj.Groups(3).Signals(4).Name = 'Yaw'
      | sbobj.Groups(3).Signals(4).XData = [0 500]
      | sbobj.Groups(3).Signals(4).YData = [0 0]
      | sbobj.Groups(3).TimeRange = [0 500]
      | sbobj.Groups(4).Name = 'ZERO'
      | sbobj.Groups(4).Signals(1).Name = 'Z'
      | sbobj.Groups(4).Signals(1).XData = [0 200]
      | sbobj.Groups(4).Signals(1).YData = [0 0]
      | sbobj.Groups(4).Signals(2).Name = 'roll'
      | sbobj.Groups(4).Signals(2).XData = [0 200]
      | sbobj.Groups(4).Signals(2).YData = [0 0]
      | sbobj.Groups(4).Signals(3).Name = 'pitch'
      | sbobj.Groups(4).Signals(3).XData = [0 200]
      | sbobj.Groups(4).Signals(3).YData = [0 0]
      | sbobj.Groups(4).Signals(4).Name = 'Yaw'
      | sbobj.Groups(4).Signals(4).XData = [0 200]
      | sbobj.Groups(4).Signals(4).YData = [0 0]
      | sbobj.Groups(4).TimeRange = [0 200]
      | sbobj.Groups(5).Name = 'SEARCH_P1'
      | sbobj.Groups(5).Signals(1).Name = 'Z'
      | sbobj.Groups(5).Signals(1).XData = [0 5 5 10 10 15 15 20 20 25 30 30 35 40 40 45 45 50 50 55 55 60 60 65 65 70 70 75 75 80 80 85 85 90 90 95 95 100 100 105 105 110 110 115 115 120 120 125 125 130 130 135 135 140 140 145 145 150 150 155 155 160 160 165 165 170 170 175 175 180 180 185 185 190 190 195 195 200]
      | sbobj.Groups(5).Signals(1).YData = [0 0 0.9 0.9 2 2 4.1 4.1 0 0 0 4 4 4 2 2 0 0 2 2 0 0 2 2 0 0 2 2 0 0 2 2 0 0 2 2 0 0 2 2 0 0 2 2 0 0 2 2 0 0 2 2 0 0 2 2 0 0 2 2 0 0 2 2 0 0 2 2 0 0 2 2 0 0 2 2 0 0]
      | sbobj.Groups(5).Signals(2).Name = 'roll'
      | sbobj.Groups(5).Signals(2).XData = [0 200]
      | sbobj.Groups(5).Signals(2).YData = [0 0]
      | sbobj.Groups(5).Signals(3).Name = 'pitch'
      | sbobj.Groups(5).Signals(3).XData = [0 200]
      | sbobj.Groups(5).Signals(3).YData = [0 0]
      | sbobj.Groups(5).Signals(4).Name = 'Yaw'
      | sbobj.Groups(5).Signals(4).XData = [0 200]
      | sbobj.Groups(5).Signals(4).YData = [0 0]
      | sbobj.Groups(5).TimeRange = [0 200]
  Z : Outport  VectorParamsAs1DForOutWhenUnconnected=off
  roll : Outport  Tag=STV Outport  Port=2  VectorParamsAs1DForOutWhenUnconnected=off
  pitch : Outport  Tag=STV Outport  Port=3  VectorParamsAs1DForOutWhenUnconnected=off
  Yaw : Outport  Tag=STV Outport  Port=4
  wires:
  Demux/1 -> Z/1
  FromWs/1 -> Demux/1
  Demux/2 -> roll/1
  Demux/3 -> pitch/1
  Demux/4 -> Yaw/1

== system three_b_attitude_control_rotationMatrix/Commands/Ground ==
  Demux : Demux  Tag=STV Demux
      settings: DisplayOption=none
  FromWs : FromWorkspace  Tag=STV FromWs  VariableName=tuvar
      SigBuilderData=|
      | common.afterFinalStr = 'Extrapolate'
      | common.sampleTime = 0
      | dataSet(1).timeRange = [0 200]
      | dataSet(1).name = 'small_steps'
      | dataSet(2).timeRange = [0 200]
      | dataSet(2).name = 'zStairs_xyConstVEL'
      | dataSet(3).timeRange = [0 500]
      | dataSet(3).name = 'sineWaves'
      | dataSet(4).timeRange = [0 200]
      | dataSet(4).name = 'ZERO'
      | dataSet(5).timeRange = [0 200]
      | dataSet(5).name = 'SEARCH_P1'
      | sbobj.Name = 'Signal Builder'
      | sbobj.Groups(1).Name = 'small_steps'
      | sbobj.Groups(1).Signals(1).Name = 'Z'
      | sbobj.Groups(1).Signals(1).XData = [0 10 10.000001 20 20.000001 30 30.000001 55 200]
      | sbobj.Groups(1).Signals(1).YData = [0 0 2 2 2 2 2 2 2]
      | sbobj.Groups(1).Signals(2).Name = 'roll'
      | sbobj.Groups(1).Signals(2).XData = [0 10 10.000001 20 20.000001 30 30.000001 55 200]
      | sbobj.Groups(1).Signals(2).YData = [0 0 0 0 3 3 3 3 3]
      | sbobj.Groups(1).Signals(3).Name = 'pitch'
      | sbobj.Groups(1).Signals(3).XData = [0 10 10.000001 20 20.000001 30 30.000001 55 200]
      | sbobj.Groups(1).Signals(3).YData = [0 0 0 0 0 0 1 1 1]
      | sbobj.Groups(1).Signals(4).Name = 'Yaw'
      | sbobj.Groups(1).Signals(4).XData = [0 200]
      | sbobj.Groups(1).Signals(4).YData = [0 0]
      | sbobj.Groups(1).TimeRange = [0 200]
      | sbobj.Groups(2).Name = 'zStairs_xyConstVEL'
      | sbobj.Groups(2).Signals(1).Name = 'Z'
      | sbobj.Groups(2).Signals(1).XData = [0 10 10.000001 20 20.000001 30 30.000001 40 40.000001 55 200]
      | sbobj.Groups(2).Signals(1).YData = [0 0 1 1 2 2 1 1 0 0 0]
      | sbobj.Groups(2).Signals(2).Name = 'roll'
      | sbobj.Groups(2).Signals(2).XData = [0 10 10.000001 20 20.000001 30 30.000001 40 40.000001 55 200]
      | sbobj.Groups(2).Signals(2).YData = [0 1 1.0000001 2 2.0000001 3 3.0000001 4 4.0000001 5.5 20]
      | sbobj.Groups(2).Signals(3).Name = 'pitch'
      | sbobj.Groups(2).Signals(3).XData = [0 10 10.000001 20 20.000001 30 30.000001 40 40.000001 55 200]
      | sbobj.Groups(2).Signals(3).YData = [0 0.5 0.50000005 1 1.00000005 1.5 1.50000005 2 2.00000005 2.75 10]
      | sbobj.Groups(2).Signals(4).Name = 'Yaw'
      | sbobj.Groups(2).Signals(4).XData = [0 200]
      | sbobj.Groups(2).Signals(4).YData = [0 0]
      | sbobj.Groups(2).TimeRange = [0 200]
      | sbobj.Groups(3).Name = 'sineWaves'
      | sbobj.Groups(3).Signals(1).Name = 'Z'
      | sbobj.Groups(3).Signals(1).XData = [0 0.1 0.2 0.3 0.4 0.5 0.6 0.7 0.8 0.9 1 1.1 ... (5001 elements, 1x5001)]
      | sbobj.Groups(3).Signals(1).YData = [0 0.0314107325553 0.0627904665622 0.0941082340641 0.125333128258 0.156434333994 0.18738115819 0.218143060119 0.248689681547 0.278990876699 0.309016742004 0.338737645607 ... (5001 elements, 1x5001)]
      | sbobj.Groups(3).Signals(2).Name = 'roll'
      | sbobj.Groups(3).Signals(2).XData = [0 0.1 0.2 0.3 0.4 0.5 0.6 0.7 0.8 0.9 1 1.1 ... (5001 elements, 1x5001)]
      | sbobj.Groups(3).Signals(2).YData = [0 0.01 0.02 0.03 0.04 0.05 0.06 0.07 0.08 0.09 0.1 0.11 ... (5001 elements, 1x5001)]
      | sbobj.Groups(3).Signals(3).Name = 'pitch'
      | sbobj.Groups(3).Signals(3).XData = [0 0.1 0.2 0.3 0.4 0.5 0.6 0.7 0.8 0.9 1 1.1 ... (5001 elements, 1x5001)]
      | sbobj.Groups(3).Signals(3).YData = [0 0.0157073040455 0.0314107325553 0.04710641095 0.0627904665622 0.0784590295926 0.0941082340641 0.109734218776 0.125333128258 0.140901113717 0.156434333994 0.171928956505 ... (5001 elements, 1x5001)]
      | sbobj.Groups(3).Signals(4).Name = 'Yaw'
      | sbobj.Groups(3).Signals(4).XData = [0 500]
      | sbobj.Groups(3).Signals(4).YData = [0 0]
      | sbobj.Groups(3).TimeRange = [0 500]
      | sbobj.Groups(4).Name = 'ZERO'
      | sbobj.Groups(4).Signals(1).Name = 'Z'
      | sbobj.Groups(4).Signals(1).XData = [0 200]
      | sbobj.Groups(4).Signals(1).YData = [0 0]
      | sbobj.Groups(4).Signals(2).Name = 'roll'
      | sbobj.Groups(4).Signals(2).XData = [0 200]
      | sbobj.Groups(4).Signals(2).YData = [0 0]
      | sbobj.Groups(4).Signals(3).Name = 'pitch'
      | sbobj.Groups(4).Signals(3).XData = [0 200]
      | sbobj.Groups(4).Signals(3).YData = [0 0]
      | sbobj.Groups(4).Signals(4).Name = 'Yaw'
      | sbobj.Groups(4).Signals(4).XData = [0 200]
      | sbobj.Groups(4).Signals(4).YData = [0 0]
      | sbobj.Groups(4).TimeRange = [0 200]
      | sbobj.Groups(5).Name = 'SEARCH_P1'
      | sbobj.Groups(5).Signals(1).Name = 'Z'
      | sbobj.Groups(5).Signals(1).XData = [0 200]
      | sbobj.Groups(5).Signals(1).YData = [0 0]
      | sbobj.Groups(5).Signals(2).Name = 'roll'
      | sbobj.Groups(5).Signals(2).XData = [0 200]
      | sbobj.Groups(5).Signals(2).YData = [0 0]
      | sbobj.Groups(5).Signals(3).Name = 'pitch'
      | sbobj.Groups(5).Signals(3).XData = [0 200]
      | sbobj.Groups(5).Signals(3).YData = [0 0]
      | sbobj.Groups(5).Signals(4).Name = 'Yaw'
      | sbobj.Groups(5).Signals(4).XData = [0 200]
      | sbobj.Groups(5).Signals(4).YData = [0 0]
      | sbobj.Groups(5).TimeRange = [0 200]
  Z : Outport  VectorParamsAs1DForOutWhenUnconnected=off
  roll : Outport  Tag=STV Outport  Port=2  VectorParamsAs1DForOutWhenUnconnected=off
  pitch : Outport  Tag=STV Outport  Port=3  VectorParamsAs1DForOutWhenUnconnected=off
  Yaw : Outport  Tag=STV Outport  Port=4
  wires:
  Demux/1 -> Z/1
  FromWs/1 -> Demux/1
  Demux/2 -> roll/1
  Demux/3 -> pitch/1
  Demux/4 -> Yaw/1

== system three_b_attitude_control_rotationMatrix/Commands/Pitch ==
  Demux : Demux  Tag=STV Demux
      settings: DisplayOption=none
  FromWs : FromWorkspace  Tag=STV FromWs  VariableName=tuvar
      SigBuilderData=|
      | common.afterFinalStr = 'Extrapolate'
      | common.sampleTime = 0
      | dataSet(1).timeRange = [0 200]
      | dataSet(1).name = 'small_steps'
      | dataSet(2).timeRange = [0 200]
      | dataSet(2).name = 'zStairs_xyConstVEL'
      | dataSet(3).timeRange = [0 500]
      | dataSet(3).name = 'sineWaves'
      | dataSet(4).timeRange = [0 200]
      | dataSet(4).name = 'ZERO'
      | dataSet(5).timeRange = [0 200]
      | dataSet(5).name = 'SEARCH_P1'
      | sbobj.Name = 'Signal Builder'
      | sbobj.Groups(1).Name = 'small_steps'
      | sbobj.Groups(1).Signals(1).Name = 'Z'
      | sbobj.Groups(1).Signals(1).XData = [0 10 10.000001 20 20.000001 30 30.000001 55 200]
      | sbobj.Groups(1).Signals(1).YData = [0 0 2 2 2 2 2 2 2]
      | sbobj.Groups(1).Signals(2).Name = 'roll'
      | sbobj.Groups(1).Signals(2).XData = [0 10 10.000001 20 20.000001 30 30.000001 55 200]
      | sbobj.Groups(1).Signals(2).YData = [0 0 0 0 3 3 3 3 3]
      | sbobj.Groups(1).Signals(3).Name = 'pitch'
      | sbobj.Groups(1).Signals(3).XData = [0 10 10.000001 20 20.000001 30 30.000001 55 200]
      | sbobj.Groups(1).Signals(3).YData = [0 0 0 0 0 0 1 1 1]
      | sbobj.Groups(1).Signals(4).Name = 'Yaw'
      | sbobj.Groups(1).Signals(4).XData = [0 200]
      | sbobj.Groups(1).Signals(4).YData = [0 0]
      | sbobj.Groups(1).TimeRange = [0 200]
      | sbobj.Groups(2).Name = 'zStairs_xyConstVEL'
      | sbobj.Groups(2).Signals(1).Name = 'Z'
      | sbobj.Groups(2).Signals(1).XData = [0 10 10.000001 20 20.000001 30 30.000001 40 40.000001 55 200]
      | sbobj.Groups(2).Signals(1).YData = [0 0 1 1 2 2 1 1 0 0 0]
      | sbobj.Groups(2).Signals(2).Name = 'roll'
      | sbobj.Groups(2).Signals(2).XData = [0 10 10.000001 20 20.000001 30 30.000001 40 40.000001 55 200]
      | sbobj.Groups(2).Signals(2).YData = [0 1 1.0000001 2 2.0000001 3 3.0000001 4 4.0000001 5.5 20]
      | sbobj.Groups(2).Signals(3).Name = 'pitch'
      | sbobj.Groups(2).Signals(3).XData = [0 10 10.000001 20 20.000001 30 30.000001 40 40.000001 55 200]
      | sbobj.Groups(2).Signals(3).YData = [0 0.5 0.50000005 1 1.00000005 1.5 1.50000005 2 2.00000005 2.75 10]
      | sbobj.Groups(2).Signals(4).Name = 'Yaw'
      | sbobj.Groups(2).Signals(4).XData = [0 200]
      | sbobj.Groups(2).Signals(4).YData = [0 0]
      | sbobj.Groups(2).TimeRange = [0 200]
      | sbobj.Groups(3).Name = 'sineWaves'
      | sbobj.Groups(3).Signals(1).Name = 'Z'
      | sbobj.Groups(3).Signals(1).XData = [0 0.1 0.2 0.3 0.4 0.5 0.6 0.7 0.8 0.9 1 1.1 ... (5001 elements, 1x5001)]
      | sbobj.Groups(3).Signals(1).YData = [0 0.0314107325553 0.0627904665622 0.0941082340641 0.125333128258 0.156434333994 0.18738115819 0.218143060119 0.248689681547 0.278990876699 0.309016742004 0.338737645607 ... (5001 elements, 1x5001)]
      | sbobj.Groups(3).Signals(2).Name = 'roll'
      | sbobj.Groups(3).Signals(2).XData = [0 0.1 0.2 0.3 0.4 0.5 0.6 0.7 0.8 0.9 1 1.1 ... (5001 elements, 1x5001)]
      | sbobj.Groups(3).Signals(2).YData = [0 0.01 0.02 0.03 0.04 0.05 0.06 0.07 0.08 0.09 0.1 0.11 ... (5001 elements, 1x5001)]
      | sbobj.Groups(3).Signals(3).Name = 'pitch'
      | sbobj.Groups(3).Signals(3).XData = [0 0.1 0.2 0.3 0.4 0.5 0.6 0.7 0.8 0.9 1 1.1 ... (5001 elements, 1x5001)]
      | sbobj.Groups(3).Signals(3).YData = [0 0.0157073040455 0.0314107325553 0.04710641095 0.0627904665622 0.0784590295926 0.0941082340641 0.109734218776 0.125333128258 0.140901113717 0.156434333994 0.171928956505 ... (5001 elements, 1x5001)]
      | sbobj.Groups(3).Signals(4).Name = 'Yaw'
      | sbobj.Groups(3).Signals(4).XData = [0 500]
      | sbobj.Groups(3).Signals(4).YData = [0 0]
      | sbobj.Groups(3).TimeRange = [0 500]
      | sbobj.Groups(4).Name = 'ZERO'
      | sbobj.Groups(4).Signals(1).Name = 'Z'
      | sbobj.Groups(4).Signals(1).XData = [0 200]
      | sbobj.Groups(4).Signals(1).YData = [0 0]
      | sbobj.Groups(4).Signals(2).Name = 'roll'
      | sbobj.Groups(4).Signals(2).XData = [0 200]
      | sbobj.Groups(4).Signals(2).YData = [0 0]
      | sbobj.Groups(4).Signals(3).Name = 'pitch'
      | sbobj.Groups(4).Signals(3).XData = [0 200]
      | sbobj.Groups(4).Signals(3).YData = [0 0]
      | sbobj.Groups(4).Signals(4).Name = 'Yaw'
      | sbobj.Groups(4).Signals(4).XData = [0 200]
      | sbobj.Groups(4).Signals(4).YData = [0 0]
      | sbobj.Groups(4).TimeRange = [0 200]
      | sbobj.Groups(5).Name = 'SEARCH_P1'
      | sbobj.Groups(5).Signals(1).Name = 'Z'
      | sbobj.Groups(5).Signals(1).XData = [0 9.9 200]
      | sbobj.Groups(5).Signals(1).YData = [0 0 0]
      | sbobj.Groups(5).Signals(2).Name = 'roll'
      | sbobj.Groups(5).Signals(2).XData = [0 200]
      | sbobj.Groups(5).Signals(2).YData = [0 0]
      | sbobj.Groups(5).Signals(3).Name = 'pitch'
      | sbobj.Groups(5).Signals(3).XData = [0 0.689655172414 1.37931034483 2.06896551724 2.75862068966 3.44827586207 4.13793103448 4.8275862069 5.51724137931 6.20689655172 6.89655172414 7.58620689655 ... (291 elements, 1x291)]
      | sbobj.Groups(5).Signals(3).YData = [0 5.37426100528 10.497227539 15.1293553798 19.0540513782 22.0878011112 24.088749813 24.9633353463 24.6706630635 23.2244179954 20.6922249539 17.1924864713 ... (291 elements, 1x291)]
      | sbobj.Groups(5).Signals(4).Name = 'Yaw'
      | sbobj.Groups(5).Signals(4).XData = [0 200]
      | sbobj.Groups(5).Signals(4).YData = [0 0]
      | sbobj.Groups(5).TimeRange = [0 200]
  Z : Outport  VectorParamsAs1DForOutWhenUnconnected=off
  roll : Outport  Tag=STV Outport  Port=2  VectorParamsAs1DForOutWhenUnconnected=off
  pitch : Outport  Tag=STV Outport  Port=3  VectorParamsAs1DForOutWhenUnconnected=off
  Yaw : Outport  Tag=STV Outport  Port=4
  wires:
  Demux/4 -> Yaw/1
  Demux/3 -> pitch/1
  Demux/2 -> roll/1
  FromWs/1 -> Demux/1
  Demux/1 -> Z/1

== system three_b_attitude_control_rotationMatrix/Commands/Roll ==
  Demux : Demux  Tag=STV Demux
      settings: DisplayOption=none
  FromWs : FromWorkspace  Tag=STV FromWs  VariableName=tuvar
      SigBuilderData=|
      | common.afterFinalStr = 'Extrapolate'
      | common.sampleTime = 0
      | dataSet(1).timeRange = [0 200]
      | dataSet(1).name = 'small_steps'
      | dataSet(2).timeRange = [0 200]
      | dataSet(2).name = 'zStairs_xyConstVEL'
      | dataSet(3).timeRange = [0 500]
      | dataSet(3).name = 'sineWaves'
      | dataSet(4).timeRange = [0 200]
      | dataSet(4).name = 'ZERO'
      | dataSet(5).timeRange = [0 200]
      | dataSet(5).name = 'SEARCH_P1'
      | sbobj.Name = 'Signal Builder'
      | sbobj.Groups(1).Name = 'small_steps'
      | sbobj.Groups(1).Signals(1).Name = 'Z'
      | sbobj.Groups(1).Signals(1).XData = [0 10 10.000001 20 20.000001 30 30.000001 55 200]
      | sbobj.Groups(1).Signals(1).YData = [0 0 2 2 2 2 2 2 2]
      | sbobj.Groups(1).Signals(2).Name = 'roll'
      | sbobj.Groups(1).Signals(2).XData = [0 10 10.000001 20 20.000001 30 30.000001 55 200]
      | sbobj.Groups(1).Signals(2).YData = [0 0 0 0 3 3 3 3 3]
      | sbobj.Groups(1).Signals(3).Name = 'pitch'
      | sbobj.Groups(1).Signals(3).XData = [0 10 10.000001 20 20.000001 30 30.000001 55 200]
      | sbobj.Groups(1).Signals(3).YData = [0 0 0 0 0 0 1 1 1]
      | sbobj.Groups(1).Signals(4).Name = 'Yaw'
      | sbobj.Groups(1).Signals(4).XData = [0 200]
      | sbobj.Groups(1).Signals(4).YData = [0 0]
      | sbobj.Groups(1).TimeRange = [0 200]
      | sbobj.Groups(2).Name = 'zStairs_xyConstVEL'
      | sbobj.Groups(2).Signals(1).Name = 'Z'
      | sbobj.Groups(2).Signals(1).XData = [0 10 10.000001 20 20.000001 30 30.000001 40 40.000001 55 200]
      | sbobj.Groups(2).Signals(1).YData = [0 0 1 1 2 2 1 1 0 0 0]
      | sbobj.Groups(2).Signals(2).Name = 'roll'
      | sbobj.Groups(2).Signals(2).XData = [0 10 10.000001 20 20.000001 30 30.000001 40 40.000001 55 200]
      | sbobj.Groups(2).Signals(2).YData = [0 1 1.0000001 2 2.0000001 3 3.0000001 4 4.0000001 5.5 20]
      | sbobj.Groups(2).Signals(3).Name = 'pitch'
      | sbobj.Groups(2).Signals(3).XData = [0 10 10.000001 20 20.000001 30 30.000001 40 40.000001 55 200]
      | sbobj.Groups(2).Signals(3).YData = [0 0.5 0.50000005 1 1.00000005 1.5 1.50000005 2 2.00000005 2.75 10]
      | sbobj.Groups(2).Signals(4).Name = 'Yaw'
      | sbobj.Groups(2).Signals(4).XData = [0 200]
      | sbobj.Groups(2).Signals(4).YData = [0 0]
      | sbobj.Groups(2).TimeRange = [0 200]
      | sbobj.Groups(3).Name = 'sineWaves'
      | sbobj.Groups(3).Signals(1).Name = 'Z'
      | sbobj.Groups(3).Signals(1).XData = [0 0.1 0.2 0.3 0.4 0.5 0.6 0.7 0.8 0.9 1 1.1 ... (5001 elements, 1x5001)]
      | sbobj.Groups(3).Signals(1).YData = [0 0.0314107325553 0.0627904665622 0.0941082340641 0.125333128258 0.156434333994 0.18738115819 0.218143060119 0.248689681547 0.278990876699 0.309016742004 0.338737645607 ... (5001 elements, 1x5001)]
      | sbobj.Groups(3).Signals(2).Name = 'roll'
      | sbobj.Groups(3).Signals(2).XData = [0 0.1 0.2 0.3 0.4 0.5 0.6 0.7 0.8 0.9 1 1.1 ... (5001 elements, 1x5001)]
      | sbobj.Groups(3).Signals(2).YData = [0 0.01 0.02 0.03 0.04 0.05 0.06 0.07 0.08 0.09 0.1 0.11 ... (5001 elements, 1x5001)]
      | sbobj.Groups(3).Signals(3).Name = 'pitch'
      | sbobj.Groups(3).Signals(3).XData = [0 0.1 0.2 0.3 0.4 0.5 0.6 0.7 0.8 0.9 1 1.1 ... (5001 elements, 1x5001)]
      | sbobj.Groups(3).Signals(3).YData = [0 0.0157073040455 0.0314107325553 0.04710641095 0.0627904665622 0.0784590295926 0.0941082340641 0.109734218776 0.125333128258 0.140901113717 0.156434333994 0.171928956505 ... (5001 elements, 1x5001)]
      | sbobj.Groups(3).Signals(4).Name = 'Yaw'
      | sbobj.Groups(3).Signals(4).XData = [0 500]
      | sbobj.Groups(3).Signals(4).YData = [0 0]
      | sbobj.Groups(3).TimeRange = [0 500]
      | sbobj.Groups(4).Name = 'ZERO'
      | sbobj.Groups(4).Signals(1).Name = 'Z'
      | sbobj.Groups(4).Signals(1).XData = [0 200]
      | sbobj.Groups(4).Signals(1).YData = [0 0]
      | sbobj.Groups(4).Signals(2).Name = 'roll'
      | sbobj.Groups(4).Signals(2).XData = [0 200]
      | sbobj.Groups(4).Signals(2).YData = [0 0]
      | sbobj.Groups(4).Signals(3).Name = 'pitch'
      | sbobj.Groups(4).Signals(3).XData = [0 200]
      | sbobj.Groups(4).Signals(3).YData = [0 0]
      | sbobj.Groups(4).Signals(4).Name = 'Yaw'
      | sbobj.Groups(4).Signals(4).XData = [0 200]
      | sbobj.Groups(4).Signals(4).YData = [0 0]
      | sbobj.Groups(4).TimeRange = [0 200]
      | sbobj.Groups(5).Name = 'SEARCH_P1'
      | sbobj.Groups(5).Signals(1).Name = 'Z'
      | sbobj.Groups(5).Signals(1).XData = [0 9.9 200]
      | sbobj.Groups(5).Signals(1).YData = [0 0 0]
      | sbobj.Groups(5).Signals(2).Name = 'roll'
      | sbobj.Groups(5).Signals(2).XData = [0 0.689655172414 1.37931034483 2.06896551724 2.75862068966 3.44827586207 4.13793103448 4.8275862069 5.51724137931 6.20689655172 6.89655172414 7.58620689655 ... (291 elements, 1x291)]
      | sbobj.Groups(5).Signals(2).YData = [0 5.37426100528 10.497227539 15.1293553798 19.0540513782 22.0878011112 24.088749813 24.9633353463 24.6706630635 23.2244179954 20.6922249539 17.1924864713 ... (291 elements, 1x291)]
      | sbobj.Groups(5).Signals(3).Name = 'pitch'
      | sbobj.Groups(5).Signals(3).XData = [0 200]
      | sbobj.Groups(5).Signals(3).YData = [0 0]
      | sbobj.Groups(5).Signals(4).Name = 'Yaw'
      | sbobj.Groups(5).Signals(4).XData = [0 200]
      | sbobj.Groups(5).Signals(4).YData = [0 0]
      | sbobj.Groups(5).TimeRange = [0 200]
  Z : Outport  VectorParamsAs1DForOutWhenUnconnected=off
  roll : Outport  Tag=STV Outport  Port=2  VectorParamsAs1DForOutWhenUnconnected=off
  pitch : Outport  Tag=STV Outport  Port=3  VectorParamsAs1DForOutWhenUnconnected=off
  Yaw : Outport  Tag=STV Outport  Port=4
  wires:
  Demux/4 -> Yaw/1
  Demux/3 -> pitch/1
  Demux/2 -> roll/1
  FromWs/1 -> Demux/1
  Demux/1 -> Z/1

== system three_b_attitude_control_rotationMatrix/Commands/multisteps ==
  Demux : Demux  Tag=STV Demux
      settings: DisplayOption=none
  FromWs : FromWorkspace  Tag=STV FromWs  VariableName=tuvar
      SigBuilderData=|
      | common.afterFinalStr = 'Extrapolate'
      | common.sampleTime = 0
      | dataSet(1).timeRange = [0 200]
      | dataSet(1).name = 'small_steps'
      | dataSet(2).timeRange = [0 200]
      | dataSet(2).name = 'zStairs_xyConstVEL'
      | dataSet(3).timeRange = [0 500]
      | dataSet(3).name = 'sineWaves'
      | dataSet(4).timeRange = [0 200]
      | dataSet(4).name = 'ZERO'
      | dataSet(5).timeRange = [0 200]
      | dataSet(5).name = 'SEARCH_P1'
      | sbobj.Name = 'Signal Builder'
      | sbobj.Groups(1).Name = 'small_steps'
      | sbobj.Groups(1).Signals(1).Name = 'Z'
      | sbobj.Groups(1).Signals(1).XData = [0 10 10.000001 20 20.000001 30 30.000001 55 200]
      | sbobj.Groups(1).Signals(1).YData = [0 0 2 2 2 2 2 2 2]
      | sbobj.Groups(1).Signals(2).Name = 'roll'
      | sbobj.Groups(1).Signals(2).XData = [0 10 10.000001 20 20.000001 30 30.000001 55 200]
      | sbobj.Groups(1).Signals(2).YData = [0 0 0 0 3 3 3 3 3]
      | sbobj.Groups(1).Signals(3).Name = 'pitch'
      | sbobj.Groups(1).Signals(3).XData = [0 10 10.000001 20 20.000001 30 30.000001 55 200]
      | sbobj.Groups(1).Signals(3).YData = [0 0 0 0 0 0 1 1 1]
      | sbobj.Groups(1).Signals(4).Name = 'Yaw'
      | sbobj.Groups(1).Signals(4).XData = [0 200]
      | sbobj.Groups(1).Signals(4).YData = [0 0]
      | sbobj.Groups(1).TimeRange = [0 200]
      | sbobj.Groups(2).Name = 'zStairs_xyConstVEL'
      | sbobj.Groups(2).Signals(1).Name = 'Z'
      | sbobj.Groups(2).Signals(1).XData = [0 10 10.000001 20 20.000001 30 30.000001 40 40.000001 55 200]
      | sbobj.Groups(2).Signals(1).YData = [0 0 1 1 2 2 1 1 0 0 0]
      | sbobj.Groups(2).Signals(2).Name = 'roll'
      | sbobj.Groups(2).Signals(2).XData = [0 10 10.000001 20 20.000001 30 30.000001 40 40.000001 55 200]
      | sbobj.Groups(2).Signals(2).YData = [0 1 1.0000001 2 2.0000001 3 3.0000001 4 4.0000001 5.5 20]
      | sbobj.Groups(2).Signals(3).Name = 'pitch'
      | sbobj.Groups(2).Signals(3).XData = [0 10 10.000001 20 20.000001 30 30.000001 40 40.000001 55 200]
      | sbobj.Groups(2).Signals(3).YData = [0 0.5 0.50000005 1 1.00000005 1.5 1.50000005 2 2.00000005 2.75 10]
      | sbobj.Groups(2).Signals(4).Name = 'Yaw'
      | sbobj.Groups(2).Signals(4).XData = [0 200]
      | sbobj.Groups(2).Signals(4).YData = [0 0]
      | sbobj.Groups(2).TimeRange = [0 200]
      | sbobj.Groups(3).Name = 'sineWaves'
      | sbobj.Groups(3).Signals(1).Name = 'Z'
      | sbobj.Groups(3).Signals(1).XData = [0 0.1 0.2 0.3 0.4 0.5 0.6 0.7 0.8 0.9 1 1.1 ... (5001 elements, 1x5001)]
      | sbobj.Groups(3).Signals(1).YData = [0 0.0314107325553 0.0627904665622 0.0941082340641 0.125333128258 0.156434333994 0.18738115819 0.218143060119 0.248689681547 0.278990876699 0.309016742004 0.338737645607 ... (5001 elements, 1x5001)]
      | sbobj.Groups(3).Signals(2).Name = 'roll'
      | sbobj.Groups(3).Signals(2).XData = [0 0.1 0.2 0.3 0.4 0.5 0.6 0.7 0.8 0.9 1 1.1 ... (5001 elements, 1x5001)]
      | sbobj.Groups(3).Signals(2).YData = [0 0.01 0.02 0.03 0.04 0.05 0.06 0.07 0.08 0.09 0.1 0.11 ... (5001 elements, 1x5001)]
      | sbobj.Groups(3).Signals(3).Name = 'pitch'
      | sbobj.Groups(3).Signals(3).XData = [0 0.1 0.2 0.3 0.4 0.5 0.6 0.7 0.8 0.9 1 1.1 ... (5001 elements, 1x5001)]
      | sbobj.Groups(3).Signals(3).YData = [0 0.0157073040455 0.0314107325553 0.04710641095 0.0627904665622 0.0784590295926 0.0941082340641 0.109734218776 0.125333128258 0.140901113717 0.156434333994 0.171928956505 ... (5001 elements, 1x5001)]
      | sbobj.Groups(3).Signals(4).Name = 'Yaw'
      | sbobj.Groups(3).Signals(4).XData = [0 500]
      | sbobj.Groups(3).Signals(4).YData = [0 0]
      | sbobj.Groups(3).TimeRange = [0 500]
      | sbobj.Groups(4).Name = 'ZERO'
      | sbobj.Groups(4).Signals(1).Name = 'Z'
      | sbobj.Groups(4).Signals(1).XData = [0 200]
      | sbobj.Groups(4).Signals(1).YData = [0 0]
      | sbobj.Groups(4).Signals(2).Name = 'roll'
      | sbobj.Groups(4).Signals(2).XData = [0 200]
      | sbobj.Groups(4).Signals(2).YData = [0 0]
      | sbobj.Groups(4).Signals(3).Name = 'pitch'
      | sbobj.Groups(4).Signals(3).XData = [0 200]
      | sbobj.Groups(4).Signals(3).YData = [0 0]
      | sbobj.Groups(4).Signals(4).Name = 'Yaw'
      | sbobj.Groups(4).Signals(4).XData = [0 200]
      | sbobj.Groups(4).Signals(4).YData = [0 0]
      | sbobj.Groups(4).TimeRange = [0 200]
      | sbobj.Groups(5).Name = 'SEARCH_P1'
      | sbobj.Groups(5).Signals(1).Name = 'Z'
      | sbobj.Groups(5).Signals(1).XData = [0 7 27 32 52 57 77 82 102 107 127 132 157 187 200]
      | sbobj.Groups(5).Signals(1).YData = [0 5 5 5 5 5 5 5 5 5 5 5 5 0 0]
      | sbobj.Groups(5).Signals(2).Name = 'roll'
      | sbobj.Groups(5).Signals(2).XData = [0 7 27 32 52 57 77 82 102 107 127 132 157 187 200]
      | sbobj.Groups(5).Signals(2).YData = [0 5 25 25 5 5 25 25 5 5 25 25 0 0 0]
      | sbobj.Groups(5).Signals(3).Name = 'pitch'
      | sbobj.Groups(5).Signals(3).XData = [0 7 27 32 52 57 77 82 102 107 127 132 157 187 200]
      | sbobj.Groups(5).Signals(3).YData = [0 5 5 10 10 15 15 20 20 25 25 30 30 0 0]
      | sbobj.Groups(5).Signals(4).Name = 'Yaw'
      | sbobj.Groups(5).Signals(4).XData = [0 7 27 32 52 57 77 82 102 107 127 132 157 187 200]
      | sbobj.Groups(5).Signals(4).YData = [0 5 25 25 5 5 25 25 5 5 25 25 0 0 0]
      | sbobj.Groups(5).TimeRange = [0 200]
  Z : Outport  VectorParamsAs1DForOutWhenUnconnected=off
  roll : Outport  Tag=STV Outport  Port=2  VectorParamsAs1DForOutWhenUnconnected=off
  pitch : Outport  Tag=STV Outport  Port=3  VectorParamsAs1DForOutWhenUnconnected=off
  Yaw : Outport  Tag=STV Outport  Port=4
  wires:
  Demux/1 -> Z/1
  FromWs/1 -> Demux/1
  Demux/2 -> roll/1
  Demux/3 -> pitch/1
  Demux/4 -> Yaw/1

== system three_b_attitude_control_rotationMatrix/Commands/yaw ==
  Demux : Demux  Tag=STV Demux
      settings: DisplayOption=none
  FromWs : FromWorkspace  Tag=STV FromWs  VariableName=tuvar
      SigBuilderData=|
      | common.afterFinalStr = 'Extrapolate'
      | common.sampleTime = 0
      | dataSet(1).timeRange = [0 200]
      | dataSet(1).name = 'small_steps'
      | dataSet(2).timeRange = [0 200]
      | dataSet(2).name = 'zStairs_xyConstVEL'
      | dataSet(3).timeRange = [0 500]
      | dataSet(3).name = 'sineWaves'
      | dataSet(4).timeRange = [0 200]
      | dataSet(4).name = 'ZERO'
      | dataSet(5).timeRange = [0 200]
      | dataSet(5).name = 'SEARCH_P1'
      | sbobj.Name = 'Signal Builder'
      | sbobj.Groups(1).Name = 'small_steps'
      | sbobj.Groups(1).Signals(1).Name = 'Z'
      | sbobj.Groups(1).Signals(1).XData = [0 10 10.000001 20 20.000001 30 30.000001 55 200]
      | sbobj.Groups(1).Signals(1).YData = [0 0 2 2 2 2 2 2 2]
      | sbobj.Groups(1).Signals(2).Name = 'roll'
      | sbobj.Groups(1).Signals(2).XData = [0 10 10.000001 20 20.000001 30 30.000001 55 200]
      | sbobj.Groups(1).Signals(2).YData = [0 0 0 0 3 3 3 3 3]
      | sbobj.Groups(1).Signals(3).Name = 'pitch'
      | sbobj.Groups(1).Signals(3).XData = [0 10 10.000001 20 20.000001 30 30.000001 55 200]
      | sbobj.Groups(1).Signals(3).YData = [0 0 0 0 0 0 1 1 1]
      | sbobj.Groups(1).Signals(4).Name = 'Yaw'
      | sbobj.Groups(1).Signals(4).XData = [0 200]
      | sbobj.Groups(1).Signals(4).YData = [0 0]
      | sbobj.Groups(1).TimeRange = [0 200]
      | sbobj.Groups(2).Name = 'zStairs_xyConstVEL'
      | sbobj.Groups(2).Signals(1).Name = 'Z'
      | sbobj.Groups(2).Signals(1).XData = [0 10 10.000001 20 20.000001 30 30.000001 40 40.000001 55 200]
      | sbobj.Groups(2).Signals(1).YData = [0 0 1 1 2 2 1 1 0 0 0]
      | sbobj.Groups(2).Signals(2).Name = 'roll'
      | sbobj.Groups(2).Signals(2).XData = [0 10 10.000001 20 20.000001 30 30.000001 40 40.000001 55 200]
      | sbobj.Groups(2).Signals(2).YData = [0 1 1.0000001 2 2.0000001 3 3.0000001 4 4.0000001 5.5 20]
      | sbobj.Groups(2).Signals(3).Name = 'pitch'
      | sbobj.Groups(2).Signals(3).XData = [0 10 10.000001 20 20.000001 30 30.000001 40 40.000001 55 200]
      | sbobj.Groups(2).Signals(3).YData = [0 0.5 0.50000005 1 1.00000005 1.5 1.50000005 2 2.00000005 2.75 10]
      | sbobj.Groups(2).Signals(4).Name = 'Yaw'
      | sbobj.Groups(2).Signals(4).XData = [0 200]
      | sbobj.Groups(2).Signals(4).YData = [0 0]
      | sbobj.Groups(2).TimeRange = [0 200]
      | sbobj.Groups(3).Name = 'sineWaves'
      | sbobj.Groups(3).Signals(1).Name = 'Z'
      | sbobj.Groups(3).Signals(1).XData = [0 0.1 0.2 0.3 0.4 0.5 0.6 0.7 0.8 0.9 1 1.1 ... (5001 elements, 1x5001)]
      | sbobj.Groups(3).Signals(1).YData = [0 0.0314107325553 0.0627904665622 0.0941082340641 0.125333128258 0.156434333994 0.18738115819 0.218143060119 0.248689681547 0.278990876699 0.309016742004 0.338737645607 ... (5001 elements, 1x5001)]
      | sbobj.Groups(3).Signals(2).Name = 'roll'
      | sbobj.Groups(3).Signals(2).XData = [0 0.1 0.2 0.3 0.4 0.5 0.6 0.7 0.8 0.9 1 1.1 ... (5001 elements, 1x5001)]
      | sbobj.Groups(3).Signals(2).YData = [0 0.01 0.02 0.03 0.04 0.05 0.06 0.07 0.08 0.09 0.1 0.11 ... (5001 elements, 1x5001)]
      | sbobj.Groups(3).Signals(3).Name = 'pitch'
      | sbobj.Groups(3).Signals(3).XData = [0 0.1 0.2 0.3 0.4 0.5 0.6 0.7 0.8 0.9 1 1.1 ... (5001 elements, 1x5001)]
      | sbobj.Groups(3).Signals(3).YData = [0 0.0157073040455 0.0314107325553 0.04710641095 0.0627904665622 0.0784590295926 0.0941082340641 0.109734218776 0.125333128258 0.140901113717 0.156434333994 0.171928956505 ... (5001 elements, 1x5001)]
      | sbobj.Groups(3).Signals(4).Name = 'Yaw'
      | sbobj.Groups(3).Signals(4).XData = [0 500]
      | sbobj.Groups(3).Signals(4).YData = [0 0]
      | sbobj.Groups(3).TimeRange = [0 500]
      | sbobj.Groups(4).Name = 'ZERO'
      | sbobj.Groups(4).Signals(1).Name = 'Z'
      | sbobj.Groups(4).Signals(1).XData = [0 200]
      | sbobj.Groups(4).Signals(1).YData = [0 0]
      | sbobj.Groups(4).Signals(2).Name = 'roll'
      | sbobj.Groups(4).Signals(2).XData = [0 200]
      | sbobj.Groups(4).Signals(2).YData = [0 0]
      | sbobj.Groups(4).Signals(3).Name = 'pitch'
      | sbobj.Groups(4).Signals(3).XData = [0 200]
      | sbobj.Groups(4).Signals(3).YData = [0 0]
      | sbobj.Groups(4).Signals(4).Name = 'Yaw'
      | sbobj.Groups(4).Signals(4).XData = [0 200]
      | sbobj.Groups(4).Signals(4).YData = [0 0]
      | sbobj.Groups(4).TimeRange = [0 200]
      | sbobj.Groups(5).Name = 'SEARCH_P1'
      | sbobj.Groups(5).Signals(1).Name = 'Z'
      | sbobj.Groups(5).Signals(1).XData = [0 9.9 200]
      | sbobj.Groups(5).Signals(1).YData = [0 0 0]
      | sbobj.Groups(5).Signals(2).Name = 'roll'
      | sbobj.Groups(5).Signals(2).XData = [0 200]
      | sbobj.Groups(5).Signals(2).YData = [0 0]
      | sbobj.Groups(5).Signals(3).Name = 'pitch'
      | sbobj.Groups(5).Signals(3).XData = [0 200]
      | sbobj.Groups(5).Signals(3).YData = [0 0]
      | sbobj.Groups(5).Signals(4).Name = 'Yaw'
      | sbobj.Groups(5).Signals(4).XData = [0 1.05263157895 2.10526315789 3.15789473684 4.21052631579 5.26315789474 6.31578947368 7.36842105263 8.42105263158 9.47368421053 10.5263157895 11.5789473684 ... (191 elements, 1x191)]
      | sbobj.Groups(5).Signals(4).YData = [0 22.7289628443 42.9948898883 58.6016534784 67.8580186158 69.7609145105 64.1041328659 51.5006737471 33.3163175126 11.5216213197 -11.5216213197 -33.3163175126 ... (191 elements, 1x191)]
      | sbobj.Groups(5).TimeRange = [0 200]
  Z : Outport  VectorParamsAs1DForOutWhenUnconnected=off
  roll : Outport  Tag=STV Outport  Port=2  VectorParamsAs1DForOutWhenUnconnected=off
  pitch : Outport  Tag=STV Outport  Port=3  VectorParamsAs1DForOutWhenUnconnected=off
  Yaw : Outport  Tag=STV Outport  Port=4
  wires:
  Demux/4 -> Yaw/1
  Demux/3 -> pitch/1
  Demux/2 -> roll/1
  FromWs/1 -> Demux/1
  Demux/1 -> Z/1

== system three_b_attitude_control_rotationMatrix/Control allocation and motor control/Ideal Actuators with allocation ==
  THRUST_CMD : Inport
  TQ_Roll_CMD : Inport  Port=2
  TQ_Pitch_CMD : Inport  Port=3
  TQ_Yaw_CMD : Inport  Port=4
  Control allocation : Subsystem
  Perfect actuators : Subsystem  VariantControl=Choice2
  Thrust : Outport
  Mx : Outport  Port=2
  My : Outport  Port=3
  Mz : Outport  Port=4
  T_actual : Outport  Port=5
  w_mot_actual : Outport  Port=6
  wires:
  Control allocation/1(w_command) -> Perfect actuators/1(w_cmd)
  THRUST_CMD/1 -> Control allocation/1(THRUST_CMD)
  TQ_Pitch_CMD/1 -> Control allocation/3(TQ_Pitch_CMD)
  TQ_Roll_CMD/1 -> Control allocation/2(TQ_Roll_CMD)
  TQ_Yaw_CMD/1 -> Control allocation/4(TQ_Yaw_CMD)
  Perfect actuators/5(T_actual) -> T_actual/1
  Perfect actuators/6(w_mot_actual) -> w_mot_actual/1
  Perfect actuators/3(My) -> My/1
  Perfect actuators/2(Mx) -> Mx/1
  Perfect actuators/4(Mz) -> Mz/1
  Perfect actuators/1(Thrust) -> Thrust/1

== system three_b_attitude_control_rotationMatrix/Control allocation and motor control/Ideal Actuattion (direct transfer) ==
  THRUST_CMD : Inport
  TQ_Roll_CMD : Inport  Port=2
  TQ_Pitch_CMD : Inport  Port=3
  TQ_Yaw_CMD : Inport  Port=4
  Mux : Mux
  Zero : Constant  Value=[0;0;0;0]  OutDataTypeStr=Inherit: Inherit via back propagation
  Thrust : Outport
  Mx : Outport  Port=2
  My : Outport  Port=3
  Mz : Outport  Port=4
  T_actual : Outport  Port=5
  w_mot_actual : Outport  Port=6
  wires:
  Zero/1 -> w_mot_actual/1
  TQ_Pitch_CMD/1 -> Mux/3, My/1
  TQ_Roll_CMD/1 -> Mux/2, Mx/1
  TQ_Yaw_CMD/1 -> Mux/4, Mz/1
  THRUST_CMD/1 -> Mux/1, Thrust/1
  Mux/1 -> T_actual/1

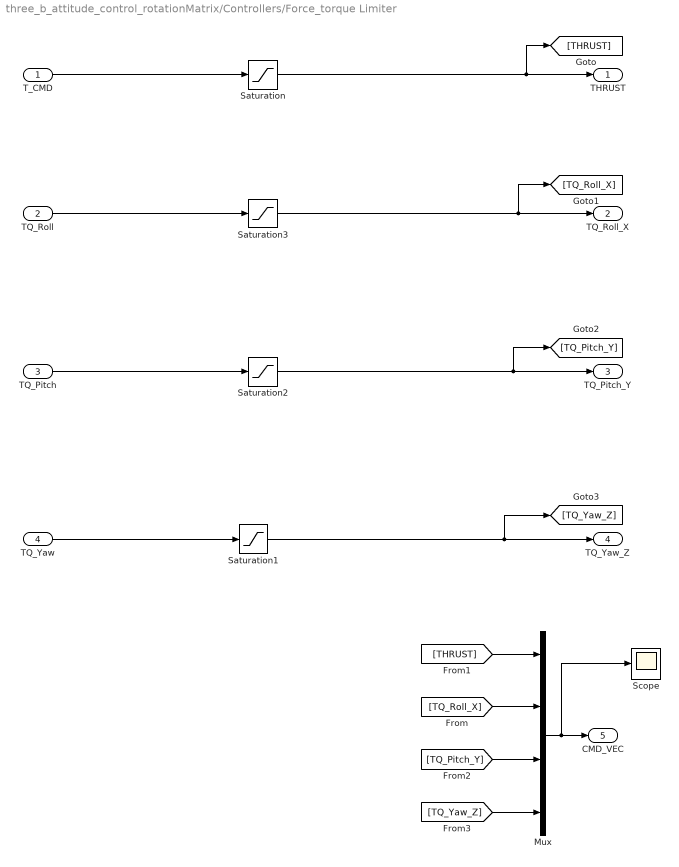
== system three_b_attitude_control_rotationMatrix/Controllers/Force_torque Limiter ==
  T_CMD : Inport
  TQ_Roll : Inport  Port=2
  TQ_Pitch : Inport  Port=3
  TQ_Yaw : Inport  Port=4
  Mux : Mux
  Saturation : Saturate  UpperLimit=4*thrust_max  LowerLimit=-4*thrust_max
      settings: AttributesFormatString=|
      | MAX =    %<UpperLimit>
      | MIN = %<LowerLimit>
  Saturation1 : Saturate  UpperLimit=2*TQ_max_per_motor  LowerLimit=-2*TQ_max_per_motor
      settings: AttributesFormatString=|
      | MAX =    %<UpperLimit>
      | MIN = %<LowerLimit>
  Saturation2 : Saturate  UpperLimit="thrust_max *  L"  LowerLimit=-thrust_max *L
      settings: AttributesFormatString=|
      | MAX =    %<UpperLimit>
      | MIN = %<LowerLimit>
  Saturation3 : Saturate  UpperLimit=thrust_max *L  LowerLimit=-thrust_max *L
      settings: AttributesFormatString=|
      | MAX =    %<UpperLimit>
      | MIN = %<LowerLimit>
  Scope : Scope
  THRUST : Outport  VectorParamsAs1DForOutWhenUnconnected=off
  TQ_Roll_X : Outport  Port=2  VectorParamsAs1DForOutWhenUnconnected=off
  TQ_Pitch_Y : Outport  Port=3  VectorParamsAs1DForOutWhenUnconnected=off
  TQ_Yaw_Z : Outport  Port=4  VectorParamsAs1DForOutWhenUnconnected=off
  CMD_VEC : Outport  Port=5  VectorParamsAs1DForOutWhenUnconnected=off
  wires:
  TQ_Yaw/1 -> Saturation1/1
  T_CMD/1 -> Saturation/1
  TQ_Pitch/1 -> Saturation2/1
  TQ_Roll/1 -> Saturation3/1
  Saturation/1 -> [THRUST], THRUST/1
  Saturation3/1 -> [TQ_Roll_X], TQ_Roll_X/1
  Saturation2/1 -> [TQ_Pitch_Y], TQ_Pitch_Y/1
  Saturation1/1 -> [TQ_Yaw_Z], TQ_Yaw_Z/1
  Mux/1 -> Scope/1, CMD_VEC/1
  [THRUST] -> Mux/1
  [TQ_Roll_X] -> Mux/2
  [TQ_Pitch_Y] -> Mux/3
  [TQ_Yaw_Z] -> Mux/4

== system three_b_attitude_control_rotationMatrix/Controllers/Rate controller ==
  w_d : Inport
  w : Inport  Port=2
  w_dot : Inport  Port=3
  Kd_rates : Gain  Gain=0.1
  Kp_rates : Gain  Gain=5
  Scope : Scope  NumInputPorts=2
  Sum : Sum  Inputs=|+-
  Sum1 : Sum  Inputs=|+-
  torques : Outport
  wires:
  Sum1/1 -> Kp_rates/1
  Sum/1 -> torques/1  "torques"
  Kp_rates/1 -> Sum/1
  Kd_rates/1 -> Sum/2  "w_d"
  w_d/1 -> Scope/1, Sum1/1
  w/1 -> Scope/2, Sum1/2
  w_dot/1 -> Kd_rates/1

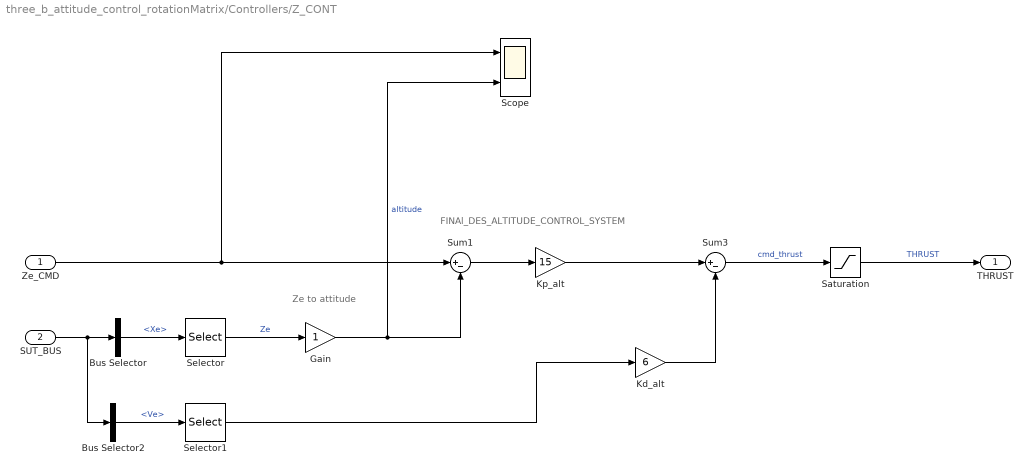
== system three_b_attitude_control_rotationMatrix/Controllers/Z_CONT ==
  note: FINAl_DES_ALTITUDE_CONTROL_SYSTEM
  note: Ze to attitude
  Ze_CMD : Inport
  SUT_BUS : Inport  Port=2
  Bus Selector : BusSelector  OutputSignals=Xe
  Bus Selector2 : BusSelector  OutputSignals=Ve
  Gain : Gain
  Kd_alt : Gain  Gain=6
  Kp_alt : Gain  Gain=15
  Saturation : Saturate  UpperLimit=4*thrust_max  LowerLimit=-4*thrust_max
  Scope : Scope  NumInputPorts=2
  Selector : Selector  InputPortWidth=3  IndexOptions=Index vector (dialog)  Indices=3  OutputSizes=1
  Selector1 : Selector  InputPortWidth=3  IndexOptions=Index vector (dialog)  Indices=3  OutputSizes=1
  Sum1 : Sum  Inputs=|+-
  Sum3 : Sum  Inputs=|+-
  THRUST : Outport  VectorParamsAs1DForOutWhenUnconnected=off
  wires:
  Gain/1 -> Sum1/2, Scope/2  "altitude"
  SUT_BUS/1 -> Bus Selector2/1, Bus Selector/1
  Bus Selector2/1 -> Selector1/1  "<Ve>"
  Bus Selector/1 -> Selector/1  "<Xe>"
  Selector/1 -> Gain/1  "Ze"
  Kd_alt/1 -> Sum3/2
  Selector1/1 -> Kd_alt/1
  Kp_alt/1 -> Sum3/1
  Saturation/1 -> THRUST/1  "THRUST"
  Sum3/1 -> Saturation/1  "cmd_thrust"
  Ze_CMD/1 -> Sum1/1, Scope/1
  Sum1/1 -> Kp_alt/1

== system three_b_attitude_control_rotationMatrix/FM_EYES/FM_Mux ==
  FM_CMD : Inport
  FM : Inport  Port=2
  Demux1 : Demux
  Demux2 : Demux
  Mux{,1..3} (4 alike) : Mux  Inputs=2
  Scope : Scope
  Scope1 : Scope
  Y1 : Outport  VectorParamsAs1DForOutWhenUnconnected=off
  Y2 : Outport  Port=2  VectorParamsAs1DForOutWhenUnconnected=off
  w3 : Outport  Port=3  VectorParamsAs1DForOutWhenUnconnected=off
  Y4 : Outport  Port=4  VectorParamsAs1DForOutWhenUnconnected=off
  wires:
  FM_CMD/1 -> Scope/1, Demux2/1
  FM/1 -> Scope1/1, Demux1/1
  Mux/1 -> Y1/1
  Mux1/1 -> Y2/1
  Mux3/1 -> Y4/1
  Mux2/1 -> w3/1
  Demux2/1 -> Mux/1
  Demux2/2 -> Mux1/1
  Demux2/3 -> Mux2/1
  Demux2/4 -> Mux3/1
  Demux1/1 -> Mux/2
  Demux1/2 -> Mux1/2
  Demux1/3 -> Mux2/2
  Demux1/4 -> Mux3/2

== system three_b_attitude_control_rotationMatrix/Quad_EOM/Gravity_G_to_B ==
  note: F_B = ^BR_G * F_G
  bRg : Inport
  Product : Product  Multiplication=Matrix(*)
  Product1 : Product
  gravity vector in inertial frame : Constant  Value=[0;0;g]  VectorParams1D=off
  mass : Constant  Value=m
  Fb_gravity : Outport  VectorParamsAs1DForOutWhenUnconnected=off
  wires:
  bRg/1 -> Product/1
  Product/1 -> Fb_gravity/1  "F_garvity in body frame"
  Product1/1 -> Product/2  "m*g"
  gravity vector in inertial frame/1 -> Product1/1  "Fg"
  mass/1 -> Product1/2

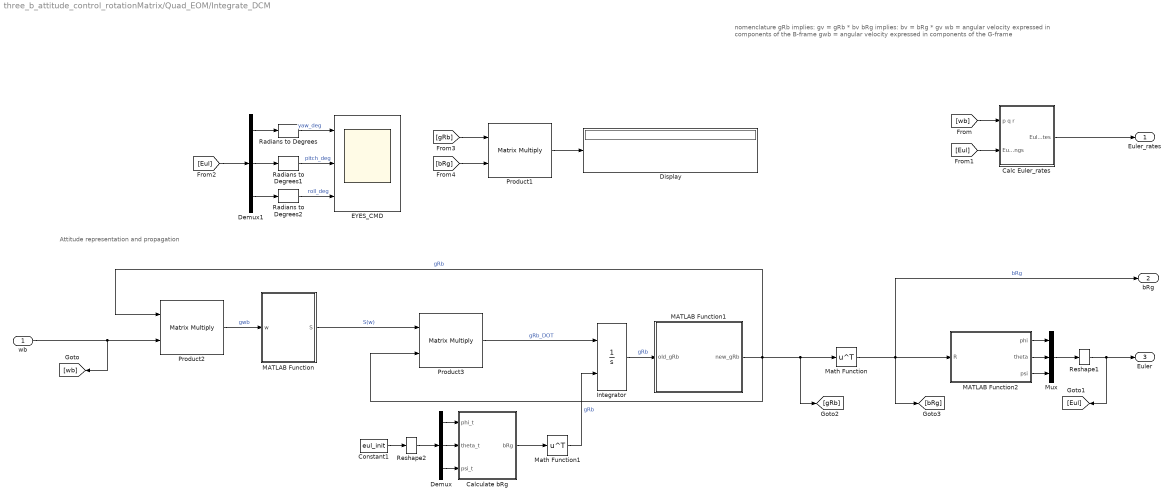
== system three_b_attitude_control_rotationMatrix/Quad_EOM/Integrate_DCM ==
  note: Attitude representation and propagation
  note: nomenclature
      | gRb implies: gv = gRb * bv
      | bRg implies: bv = bRg * gv
      |
      | wb = angular velocity expressed in components of the B-frame
      | gwb = angular velocity expressed in components of the G-frame
  wb : Inport
  Calc Euler_rates : Subsystem
  Calculate bRg : MATLAB Function  TreatAsAtomicUnit=on
  Constant1 : Constant  Value=eul_init  OutDataTypeStr=Inherit: Inherit via back propagation
  Demux : Demux  Outputs=3
  Demux1 : Demux  Outputs=3
  Display : Display
  EYES_CMD : Scope  NumInputPorts=3
  Integrator : Integrator  InitialConditionSource=external
  MATLAB Function : MATLAB Function  TreatAsAtomicUnit=on
  MATLAB Function1 : MATLAB Function  TreatAsAtomicUnit=on
  MATLAB Function2 : MATLAB Function  TreatAsAtomicUnit=on
  Math Function : Math  Operator=transpose  SignedPower=on  SaturateOnIntegerOverflow=on
  Math Function1 : Math  Operator=transpose  SignedPower=on  SaturateOnIntegerOverflow=on
  Mux : Mux  Inputs=3
  Product1 : Product  Multiplication=Matrix(*)
  Product2 : Product  Multiplication=Matrix(*)
  Product3 : Product  Multiplication=Matrix(*)
  Radians to Degrees : simulink_extras/Transformations/Radians to Degrees
  Radians to Degrees1 : simulink_extras/Transformations/Radians to Degrees
  Radians to Degrees2 : simulink_extras/Transformations/Radians to Degrees
  Reshape1 : Reshape  OutputDimensionality=Column vector (2-D)
  Reshape2 : Reshape  OutputDimensionality=Column vector (2-D)
  Euler_rates : Outport
  bRg : Outport  Port=2
  Euler : Outport  Port=3
  wires:
  MATLAB Function1/1(new_gRb) -> Product3/2, Product2/1, Math Function/1, [gRb]  "gRb"
  [bRg] -> Product1/2
  [gRb] -> Product1/1
  Product2/1 -> MATLAB Function/1(w)  "gwb"
  Calc Euler_rates/1(Euler_rates) -> Euler_rates/1
  [Eul] -> Demux1/1
  Demux1/2 -> Radians to Degrees1/1
  Demux1/3 -> Radians to Degrees2/1
  Radians to Degrees2/1 -> EYES_CMD/3  "roll_deg"
  Radians to Degrees1/1 -> EYES_CMD/2  "pitch_deg"
  Radians to Degrees/1 -> EYES_CMD/1  "yaw_deg"
  Demux1/1 -> Radians to Degrees/1
  Product1/1 -> Display/1
  [Eul] -> Calc Euler_rates/2(Euler_angs)
  [wb] -> Calc Euler_rates/1("p q r ")
  Reshape1/1 -> [Eul], Euler/1
  Mux/1 -> Reshape1/1
  Reshape2/1 -> Demux/1
  Constant1/1 -> Reshape2/1
  Calculate bRg/1(bRg) -> Math Function1/1
  Demux/2 -> Calculate bRg/2(theta_t)
  Demux/1 -> Calculate bRg/1(phi_t)
  Math Function1/1 -> Integrator/2  "gRb"
  Demux/3 -> Calculate bRg/3(psi_t)
  wb/1 -> Product2/2, [wb]
  MATLAB Function2/3(psi) -> Mux/3
  MATLAB Function2/2(theta) -> Mux/2
  MATLAB Function2/1(phi) -> Mux/1
  Product3/1 -> Integrator/1  "gRb_DOT"
  Integrator/1 -> MATLAB Function1/1(old_gRb)  "gRb"
  Math Function/1 -> [bRg], bRg/1, MATLAB Function2/1(R)  "bRg"
  MATLAB Function/1(S) -> Product3/1  "S(w)"

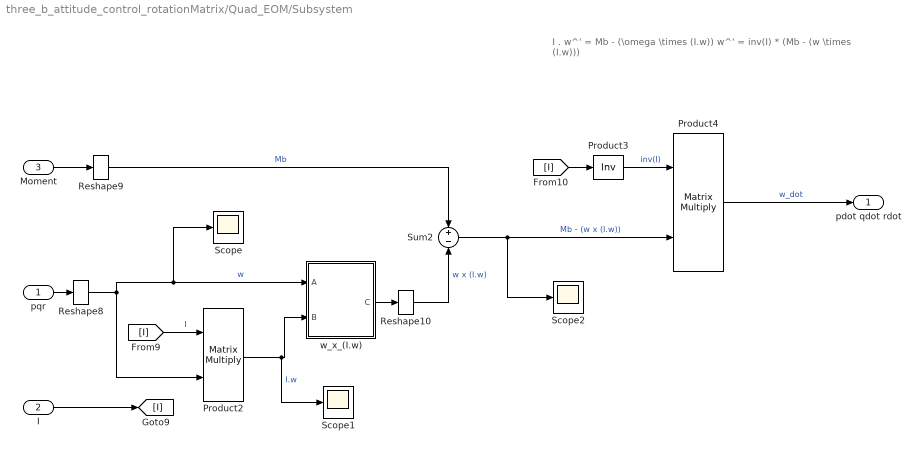
== system three_b_attitude_control_rotationMatrix/Quad_EOM/Subsystem ==
  note: I . w^' = Mb - (\omega \times (I.w))
      |
      | w^' = inv(I) * (Mb - (w \times (I.w)))
  pqr : Inport
  I : Inport  Port=2
  Moment : Inport  Port=3
  Product2 : Product  Multiplication=Matrix(*)  InputSameDT=on  SaturateOnIntegerOverflow=on  OutDataTypeStr=Inherit: Same as first input
  Product3 : Product  Inputs=/  Multiplication=Matrix(*)  SaturateOnIntegerOverflow=on  OutDataTypeStr=Inherit: Same as first input
  Product4 : Product  Multiplication=Matrix(*)  SaturateOnIntegerOverflow=on  OutDataTypeStr=Inherit: Same as first input
  Reshape10 : Reshape  OutputDimensionality=Column vector (2-D)
  Reshape8 : Reshape  OutputDimensionality=Column vector (2-D)
  Reshape9 : Reshape  OutputDimensionality=Column vector (2-D)
  Scope : Scope
  Scope1 : Scope
  Scope2 : Scope
  Sum2 : Sum  Inputs=+|-  SaturateOnIntegerOverflow=on
  w_x_(I.w) : Subsystem
      mask Display:
      | text(.5,.5,'Cross\nProduct\n\nC = AxB', ...
      | 	'HorizontalAlignment','Center',...
      | 	'VerticalAlignment','middle')
  pdot qdot rdot : Outport
  wires:
  Product2/1 -> Scope1/1, w_x_(I.w)/2(B)  "I.w"
  Product3/1 -> Product4/1  "inv(I)"
  Reshape8/1 -> Scope/1, w_x_(I.w)/1(A), Product2/2  "w"
  [I] -> Product3/1
  pqr/1 -> Reshape8/1
  Reshape9/1 -> Sum2/1  "Mb"
  Sum2/1 -> Scope2/1, Product4/2  "Mb - (w x (I.w))"
  Reshape10/1 -> Sum2/2  "w x (I.w)"
  w_x_(I.w)/1(C) -> Reshape10/1
  [I] -> Product2/1  "I"
  Product4/1 -> pdot qdot rdot/1  "w_dot"
  Moment/1 -> Reshape9/1
  I/1 -> [I]

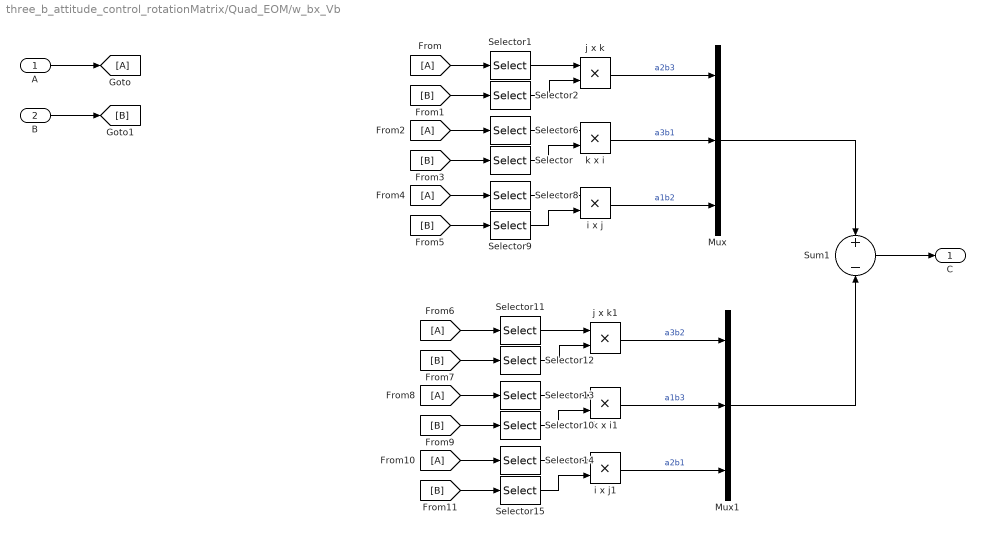
== system three_b_attitude_control_rotationMatrix/Quad_EOM/w_bx_Vb ==
  A : Inport
  B : Inport  Port=2
  Mux : Mux  Inputs=3
  Mux1 : Mux  Inputs=3
  Selector{,8,13,15} (4 alike) : Selector  InputPortWidth=3  IndexOptions=Index vector (dialog)  Indices=1  OutputSizes=1
  Selector{1,9,12,14} (4 alike) : Selector  InputPortWidth=3  IndexOptions=Index vector (dialog)  Indices=2  OutputSizes=1
  Selector{2,6,10..11} (4 alike) : Selector  InputPortWidth=3  IndexOptions=Index vector (dialog)  Indices=3  OutputSizes=1
  Sum1 : Sum  Inputs=+|-  InputSameDT=on  SaturateOnIntegerOverflow=on  OutDataTypeStr=Inherit: Same as first input
  i x j : Product  InputSameDT=on  SaturateOnIntegerOverflow=on  OutDataTypeStr=Inherit: Same as first input
  i x j1 : Product  InputSameDT=on  SaturateOnIntegerOverflow=on  OutDataTypeStr=Inherit: Same as first input
  j x k : Product  InputSameDT=on  SaturateOnIntegerOverflow=on  OutDataTypeStr=Inherit: Same as first input
  j x k1 : Product  InputSameDT=on  SaturateOnIntegerOverflow=on  OutDataTypeStr=Inherit: Same as first input
  k x i : Product  InputSameDT=on  SaturateOnIntegerOverflow=on  OutDataTypeStr=Inherit: Same as first input
  k x i1 : Product  InputSameDT=on  SaturateOnIntegerOverflow=on  OutDataTypeStr=Inherit: Same as first input
  C : Outport
  wires:
  i x j/1 -> Mux/3  "a1b2"
  k x i/1 -> Mux/2  "a3b1"
  j x k/1 -> Mux/1  "a2b3"
  Mux/1 -> Sum1/1
  Sum1/1 -> C/1
  Selector1/1 -> j x k/1
  Selector2/1 -> j x k/2
  B/1 -> [B]
  A/1 -> [A]
  [B] -> Selector2/1
  [A] -> Selector1/1
  [A] -> Selector6/1
  [B] -> Selector/1
  Selector6/1 -> k x i/1
  Selector/1 -> k x i/2
  [A] -> Selector8/1
  [B] -> Selector9/1
  Selector8/1 -> i x j/1
  Selector9/1 -> i x j/2
  i x j1/1 -> Mux1/3  "a2b1"
  k x i1/1 -> Mux1/2  "a1b3"
  j x k1/1 -> Mux1/1  "a3b2"
  Mux1/1 -> Sum1/2
  Selector11/1 -> j x k1/1
  Selector12/1 -> j x k1/2
  [B] -> Selector12/1
  [A] -> Selector11/1
  [A] -> Selector13/1
  [B] -> Selector10/1
  Selector13/1 -> k x i1/1
  Selector10/1 -> k x i1/2
  [A] -> Selector14/1
  [B] -> Selector15/1
  Selector14/1 -> i x j1/1
  Selector15/1 -> i x j1/2

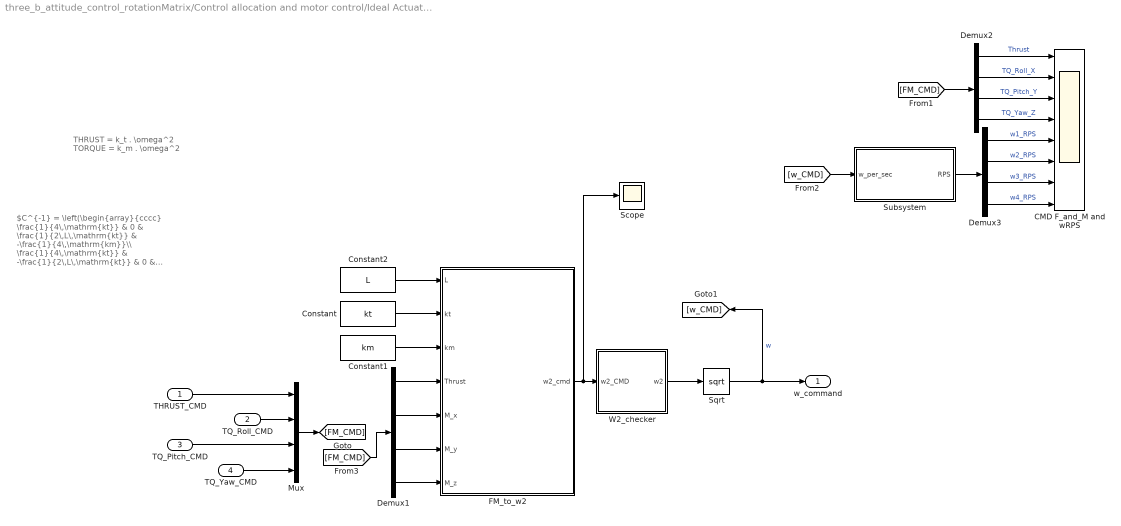
== system three_b_attitude_control_rotationMatrix/Control allocation and motor control/Ideal Actuators with allocation/Control allocation ==
  note: $C^{-1} = \left(\begin{array}{cccc} \frac{1}{4\,\mathrm{kt}} & 0 & \frac{1}{2\,L\,\mathrm{kt}} & -\frac{1}{4\,\mathrm{km}}\\ \frac{1}{4\,\mathrm{kt}} & -\frac{1}{2\,L\,\mathrm{kt}} & 0 & \frac{1}{4\,\mathrm{km}}\\ \frac{1}{4\,\mathrm{kt}} & 0 & -\frac{1}{2\,L\,\mathrm{kt}} & -\frac{1}{4\,\mathrm{km}}\\ \frac{1}{4\,\mathrm{kt}} & \frac{1}{2\,L\,\mathrm{kt}} & 0 & \frac{1}{4\,\mathrm{km}} \end{array}\right)$
  note: THRUST = k_t . \omega^2
      |
      | TORQUE = k_m . \omega^2
  THRUST_CMD : Inport
  TQ_Roll_CMD : Inport  Port=2
  TQ_Pitch_CMD : Inport  Port=3
  TQ_Yaw_CMD : Inport  Port=4
  CMD F_and_M and wRPS : Scope  NumInputPorts=8
  Constant : Constant  Value=kt
  Constant1 : Constant  Value=km
  Constant2 : Constant  Value=L
  Demux1 : Demux
  Demux2 : Demux
  Demux3 : Demux
  FM_to_w2 : MATLAB Function  TreatAsAtomicUnit=on
  Mux : Mux
  Scope : Scope
  Sqrt : Sqrt  SaturateOnIntegerOverflow=on
  Subsystem : Subsystem
  W2_checker : Subsystem
  w_command : Outport  VectorParamsAs1DForOutWhenUnconnected=off
  wires:
  Constant1/1 -> FM_to_w2/3(km)
  Constant/1 -> FM_to_w2/2(kt)
  Constant2/1 -> FM_to_w2/1(L)
  FM_to_w2/1(w2_cmd) -> Scope/1, W2_checker/1(w2_CMD)
  Sqrt/1 -> w_command/1, [w_CMD]  "w"
  W2_checker/1(w2) -> Sqrt/1
  Demux1/1 -> FM_to_w2/4(Thrust)
  Demux1/2 -> FM_to_w2/5(M_x)
  Demux1/3 -> FM_to_w2/6(M_y)
  Demux1/4 -> FM_to_w2/7(M_z)
  THRUST_CMD/1 -> Mux/1
  TQ_Roll_CMD/1 -> Mux/2
  TQ_Pitch_CMD/1 -> Mux/3
  TQ_Yaw_CMD/1 -> Mux/4
  Mux/1 -> [FM_CMD]
  [FM_CMD] -> Demux1/1
  Demux2/1 -> CMD F_and_M and wRPS/1  "Thrust"
  Demux2/2 -> CMD F_and_M and wRPS/2  "TQ_Roll_X"
  Demux2/3 -> CMD F_and_M and wRPS/3  "TQ_Pitch_Y"
  Demux2/4 -> CMD F_and_M and wRPS/4  "TQ_Yaw_Z"
  Demux3/2 -> CMD F_and_M and wRPS/6  "w2_RPS"
  Demux3/1 -> CMD F_and_M and wRPS/5  "w1_RPS"
  Demux3/4 -> CMD F_and_M and wRPS/8  "w4_RPS"
  Demux3/3 -> CMD F_and_M and wRPS/7  "w3_RPS"
  [FM_CMD] -> Demux2/1
  Subsystem/1(RPS) -> Demux3/1
  [w_CMD] -> Subsystem/1(w_per_sec)

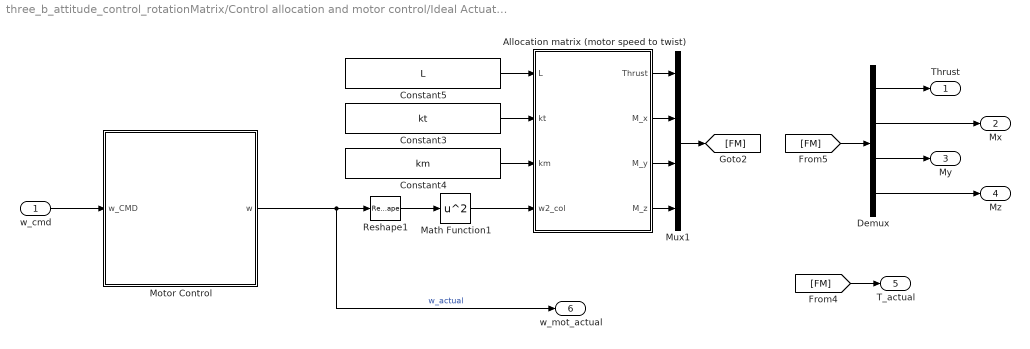
== system three_b_attitude_control_rotationMatrix/Control allocation and motor control/Ideal Actuators with allocation/Perfect actuators ==
  w_cmd : Inport
  Allocation matrix (motor speed to twist) : MATLAB Function  TreatAsAtomicUnit=on
  Constant3 : Constant  Value=kt
  Constant4 : Constant  Value=km
  Constant5 : Constant  Value=L
  Demux : Demux
  Math Function1 : Math  Operator=square  SignedPower=on  SaturateOnIntegerOverflow=on
  Motor Control : Subsystem
      mask Display: image('$imagefile'); % Use "Edit Image" on toolstrip to change.
  Mux1 : Mux
  Reshape1 : Reshape  OutputDimensionality=Column vector (2-D)
  Thrust : Outport  VectorParamsAs1DForOutWhenUnconnected=off
  Mx : Outport  Port=2  VectorParamsAs1DForOutWhenUnconnected=off
  My : Outport  Port=3  VectorParamsAs1DForOutWhenUnconnected=off
  Mz : Outport  Port=4  VectorParamsAs1DForOutWhenUnconnected=off
  T_actual : Outport  Port=5  VectorParamsAs1DForOutWhenUnconnected=off
  w_mot_actual : Outport  Port=6  VectorParamsAs1DForOutWhenUnconnected=off
  wires:
  Demux/2 -> Mx/1
  Demux/1 -> Thrust/1
  Demux/3 -> My/1
  Demux/4 -> Mz/1
  [FM] -> Demux/1
  Constant3/1 -> Allocation matrix (motor speed to twist)/2(kt)
  Mux1/1 -> [FM]
  Allocation matrix (motor speed to twist)/4(M_z) -> Mux1/4
  Allocation matrix (motor speed to twist)/1(Thrust) -> Mux1/1
  Allocation matrix (motor speed to twist)/2(M_x) -> Mux1/2
  Allocation matrix (motor speed to twist)/3(M_y) -> Mux1/3
  Constant4/1 -> Allocation matrix (motor speed to twist)/3(km)
  [FM] -> T_actual/1
  Constant5/1 -> Allocation matrix (motor speed to twist)/1(L)
  Math Function1/1 -> Allocation matrix (motor speed to twist)/4(w2_col)
  Reshape1/1 -> Math Function1/1
  Motor Control/1(w) -> w_mot_actual/1, Reshape1/1  "w_actual"
  w_cmd/1 -> Motor Control/1(w_CMD)

== system three_b_attitude_control_rotationMatrix/Quad_EOM/Integrate_DCM/Calc Euler_rates ==
  "p q r " : Inport
  Euler_angs : Inport  Port=2
  Demux1 : Demux  Outputs=3
  Demux2 : Demux  Outputs=3
  Demux3 : Demux  Outputs=3
  Mux1 : Mux  Inputs=3
  Reshape1 : Reshape  OutputDimensionality=Column vector (2-D)
  Reshape2 : Reshape  OutputDimensionality=Column vector (2-D)
  Terminator : Terminator
  euler_rates : MATLAB Function  TreatAsAtomicUnit=on
  Euler_rates : Outport
  wires:
  Demux2/2 -> Mux1/2  "thetadot_Y2_pitch"
  Demux1/1 -> euler_rates/1(phi_t)  "phi"
  Demux3/2 -> euler_rates/4(q)
  Demux2/1 -> Mux1/1  "phidot_Z1_yaw"
  "p q r "/1 -> Reshape1/1
  Euler_angs/1 -> Demux1/1
  Demux3/1 -> euler_rates/3(p)
  Reshape2/1 -> Euler_rates/1
  Reshape1/1 -> Demux3/1  "wb"
  Demux3/3 -> euler_rates/5(r)
  Demux1/3 -> Terminator/1  "psi"
  euler_rates/1(euler_rates) -> Demux2/1  "euler_rates"
  Demux1/2 -> euler_rates/2(theta_t)  "theta"
  Mux1/1 -> Reshape2/1
  Demux2/3 -> Mux1/3  "psidot_X3_roll"

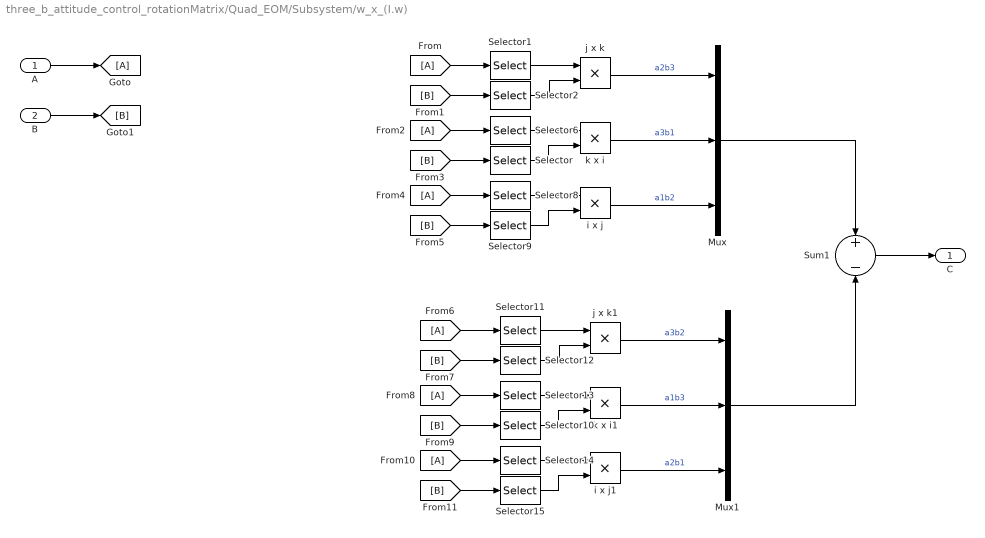
== system three_b_attitude_control_rotationMatrix/Quad_EOM/Subsystem/w_x_(I.w) ==
  A : Inport
  B : Inport  Port=2
  Mux : Mux  Inputs=3
  Mux1 : Mux  Inputs=3
  Selector{,8,13,15} (4 alike) : Selector  InputPortWidth=3  IndexOptions=Index vector (dialog)  Indices=1  OutputSizes=1
  Selector{1,9,12,14} (4 alike) : Selector  InputPortWidth=3  IndexOptions=Index vector (dialog)  Indices=2  OutputSizes=1
  Selector{2,6,10..11} (4 alike) : Selector  InputPortWidth=3  IndexOptions=Index vector (dialog)  Indices=3  OutputSizes=1
  Sum1 : Sum  Inputs=+|-  InputSameDT=on  SaturateOnIntegerOverflow=on  OutDataTypeStr=Inherit: Same as first input
  i x j : Product  InputSameDT=on  SaturateOnIntegerOverflow=on  OutDataTypeStr=Inherit: Same as first input
  i x j1 : Product  InputSameDT=on  SaturateOnIntegerOverflow=on  OutDataTypeStr=Inherit: Same as first input
  j x k : Product  InputSameDT=on  SaturateOnIntegerOverflow=on  OutDataTypeStr=Inherit: Same as first input
  j x k1 : Product  InputSameDT=on  SaturateOnIntegerOverflow=on  OutDataTypeStr=Inherit: Same as first input
  k x i : Product  InputSameDT=on  SaturateOnIntegerOverflow=on  OutDataTypeStr=Inherit: Same as first input
  k x i1 : Product  InputSameDT=on  SaturateOnIntegerOverflow=on  OutDataTypeStr=Inherit: Same as first input
  C : Outport
  wires:
  i x j/1 -> Mux/3  "a1b2"
  k x i/1 -> Mux/2  "a3b1"
  j x k/1 -> Mux/1  "a2b3"
  Mux/1 -> Sum1/1
  Sum1/1 -> C/1
  Selector1/1 -> j x k/1
  Selector2/1 -> j x k/2
  B/1 -> [B]
  A/1 -> [A]
  [B] -> Selector2/1
  [A] -> Selector1/1
  [A] -> Selector6/1
  [B] -> Selector/1
  Selector6/1 -> k x i/1
  Selector/1 -> k x i/2
  [A] -> Selector8/1
  [B] -> Selector9/1
  Selector8/1 -> i x j/1
  Selector9/1 -> i x j/2
  i x j1/1 -> Mux1/3  "a2b1"
  k x i1/1 -> Mux1/2  "a1b3"
  j x k1/1 -> Mux1/1  "a3b2"
  Mux1/1 -> Sum1/2
  Selector11/1 -> j x k1/1
  Selector12/1 -> j x k1/2
  [B] -> Selector12/1
  [A] -> Selector11/1
  [A] -> Selector13/1
  [B] -> Selector10/1
  Selector13/1 -> k x i1/1
  Selector10/1 -> k x i1/2
  [A] -> Selector14/1
  [B] -> Selector15/1
  Selector14/1 -> i x j1/1
  Selector15/1 -> i x j1/2

== system three_b_attitude_control_rotationMatrix/Control allocation and motor control/Ideal Actuators with allocation/Control allocation/Subsystem ==
  w_per_sec : Inport
  Constant3 : Constant  Value=3.141592653589793
  Gain1 : Gain  Gain=2
  Product : Product  Inputs=*/
  RPS : Outport
  wires:
  Gain1/1 -> Product/2  "2PI"
  w_per_sec/1 -> Product/1
  Constant3/1 -> Gain1/1
  Product/1 -> RPS/1

== system three_b_attitude_control_rotationMatrix/Control allocation and motor control/Ideal Actuators with allocation/Control allocation/W2_checker ==
  w2_CMD : Inport
  Assertion{,1..3} (4 alike) : Assertion
  Compare To Constant : simulink/Logic and Bit Operations/Compare To Constant  relop=>=  const=0  OutDataTypeStr=boolean
  Demux : Demux
  w2 : Outport  VectorParamsAs1DForOutWhenUnconnected=off
  wires:
  w2_CMD/1 -> w2/1, Compare To Constant/1
  Compare To Constant/1 -> Demux/1
  Demux/1 -> Assertion/1
  Demux/4 -> Assertion3/1
  Demux/3 -> Assertion2/1
  Demux/2 -> Assertion1/1

== system three_b_attitude_control_rotationMatrix/Control allocation and motor control/Ideal Actuators with allocation/Perfect actuators/Motor Control ==
  w_CMD : Inport
  Demux : Demux
  Mux : Mux
  w CMD vs Actual : Scope  NumInputPorts=4
  w_MUX : Subsystem
  w : Outport  VectorParamsAs1DForOutWhenUnconnected=off
  wires:
  Demux/4 -> Mux/4
  Demux/3 -> Mux/3
  Demux/2 -> Mux/2
  Demux/1 -> Mux/1
  w_CMD/1 -> [W_CMD], Demux/1
  w_MUX/4(w4) -> w CMD vs Actual/4
  w_MUX/2(w2) -> w CMD vs Actual/2
  w_MUX/3(w3) -> w CMD vs Actual/3
  w_MUX/1(w1) -> w CMD vs Actual/1
  [W_CMD] -> w_MUX/1(W_CMD)
  Mux/1 -> w_MUX/2(W), w/1

== system three_b_attitude_control_rotationMatrix/Control allocation and motor control/Ideal Actuators with allocation/Perfect actuators/Motor Control/w_MUX ==
  W_CMD : Inport
  W : Inport  Port=2
  Demux1 : Demux
  Demux2 : Demux
  Mux{,1..3} (4 alike) : Mux  Inputs=2
  w1 : Outport  VectorParamsAs1DForOutWhenUnconnected=off
  w2 : Outport  Port=2  VectorParamsAs1DForOutWhenUnconnected=off
  w3 : Outport  Port=3  VectorParamsAs1DForOutWhenUnconnected=off
  w4 : Outport  Port=4  VectorParamsAs1DForOutWhenUnconnected=off
  wires:
  W_CMD/1 -> Demux2/1
  W/1 -> Demux1/1
  Mux/1 -> w1/1
  Mux1/1 -> w2/1
  Mux3/1 -> w4/1
  Mux2/1 -> w3/1
  Demux2/1 -> Mux/1
  Demux2/2 -> Mux1/1
  Demux2/3 -> Mux2/1
  Demux2/4 -> Mux3/1
  Demux1/1 -> Mux/2
  Demux1/2 -> Mux1/2
  Demux1/3 -> Mux2/2
  Demux1/4 -> Mux3/2

== matlab function three_b_attitude_control_rotationMatrix/Quad_EOM/Integrate_DCM/Calculate bRg ==
  data: phi_t input; bRg output; theta_t input; psi_t input
function bRg = calc_bRg(phi_t,theta_t,psi_t)
%#codegen

%    This function was generated by the Symbolic Math Toolbox version 8.7.
%    04-Nov-2022 08:55:57

bRg = reshape([cos(psi_t).*cos(theta_t),-cos(phi_t).*sin(psi_t)+cos(psi_t).*sin(phi_t).*sin(theta_t),sin(phi_t).*sin(psi_t)+cos(phi_t).*cos(psi_t).*sin(theta_t),cos(theta_t).*sin(psi_t),cos(phi_t).*cos(psi_t)+sin(phi_t).*sin(psi_t).*sin(theta_t),-cos(psi_t).*sin(phi_t)+cos(phi_t).*sin(psi_t).*sin(theta_t),-sin(theta_t),cos(theta_t).*sin(phi_t),cos(phi_t).*cos(theta_t)],[3,3]);
